simulink model "asbdhc2(1)"  (R2024b)
settings: Solver=ode23  StartTime=0.0  StopTime=100  MaxStep=1/30  RelTol=1e-2  AbsTol=1e-3  EnableMultiTasking=on
PreLoadFcn:
  | load asbdhc2_init;
model workspace (MAT data in the model file):
  op_trim1 = opcond.OperatingReport
  op_trim1.TerminationString_ = '成功满足工作点设定。'
  op_trim1.OptimizationOutput_.iterations = 4
  op_trim1.OptimizationOutput_.funcCount = 131
  op_trim1.OptimizationOutput_.lssteplength = 1
  op_trim1.OptimizationOutput_.stepsize = 7.33681796008e-13
  op_trim1.OptimizationOutput_.algorithm = 'active-set'
  op_trim1.OptimizationOutput_.firstorderopt = 0
  op_trim1.OptimizationOutput_.constrviolation = 7.66053886991e-13
  op_trim1.OptimizationOutput_.message = '找到满足约束的局部最小值。
    | 
    | 优化已完成，因为目标函数沿
    | 可行方向在最优性容差值范围内呈现非递减，
    | 并且在约束容差值范围内满足约束。
    | 
    | <停止条件详细信息>
    | 
    | 优化已完成: 一阶最优性测度 0.000000e+00 小于
    | options.OptimalityTolerance = 1.000000e-06，并且最大约束违反值
    | 7.660539e-13 小于 options.ConstraintTolerance = 1.000000e-06。'
  op_trim1.OptimizationOutput_.bestfeasible.x = [1.78783981281e-13; -2.72791413757e-14; 0.0648890450075; 57.2809333751; -0.648532707323; 3.72213065063; 1.07573812912e-14; 6.1317224328e-16; 3.38561643998e-14; 0; 0; 0; 0; 0; 0; 0; 0; 0; 0; 0; 0; 0; 0; 0; 0; 0; 0; -0.158142456848; -0.114677786174; 0.799732063917; 0.0107264222622]
  op_trim1.OptimizationOutput_.bestfeasible.fval = 0
  op_trim1.OptimizationOutput_.bestfeasible.constrviolation = 7.66053886991e-13
  op_trim1.OptimizationOutput_.bestfeasible.firstorderopt = 0
  op_trim1.OptimizationOutput_.progress = {'<font face="monospaced"; size=3><BR>', '正在优化以求解所有所需的 dx/dt=0、x(k+1)-x(k)=0 和 y=ydes。<BR>', ' <BR>', '(最大误差)模块<BR>', ' ---------------------------------------------------------<BR>', '(1.87100e-01) asbdhc2/De Havilland Beaver Airframe/Aircraft Dynamics/6DOF (Quaternion)/ub,vb,wb<BR>', '(1.25955e-02) asbdhc2/De Havilland Beaver Airframe/Aircraft Dynamics/6DOF (Quaternion)/xe,ye,ze<BR>', '(4.14127e-06) asbdhc2/De Havilland Beaver Airframe/Aircraft Dynamics/6DOF (Quaternion)/xe,ye,ze<BR>', '(7.66054e-13) asbdhc2/De Havilland Beaver Airframe/Aircraft Dynamics/6DOF (Quaternion)/xe,ye,ze<BR>', '(7.66054e-13) asbdhc2/De Havilland Beaver Airframe/Aircraft Dynamics/6DOF (Quaternion)/xe,ye,ze<BR>', ' <BR>', '成功满足工作点设定。<BR>'}
  op_trim1.Model_ = 'asbdhc2'
  op_trim1.States_(1) = opcond.StateReport
  op_trim1.States_(1).dx_ = [0; 0; 0]
  op_trim1.States_(1).Nx_ = 3
  op_trim1.States_(1).Block_ = 'asbdhc2/De Havilland Beaver Airframe/Aircraft Dynamics/6DOF (Quaternion)/Calculate DCM &
    | Euler Angles/phi
    | theta
    | psi'
  op_trim1.States_(1).x_ = [0; 0.0648890450075; 0]
  op_trim1.States_(1).SteadyState_ = [1; 1; 1]
  op_trim1.States_(1).dxMin_ = [-Inf; -Inf; -Inf]
  op_trim1.States_(1).dxMax_ = [Inf; Inf; Inf]
  op_trim1.States_(1).Known_ = [1; 0; 1]
  op_trim1.States_(1).Min_ = [-Inf; -Inf; -Inf]
  op_trim1.States_(1).Max_ = [Inf; Inf; Inf]
  op_trim1.States_(2) = opcond.StateReport
  op_trim1.States_(2).dx_ = [-7.37914856069e-14; 2.85609872713e-14; -2.97018129939e-14]
  op_trim1.States_(2).Nx_ = 3
  op_trim1.States_(2).Block_ = 'asbdhc2/De Havilland Beaver Airframe/Aircraft Dynamics/6DOF (Quaternion)/p,q,r '
  op_trim1.States_(2).x_ = [0; 0; 0]
  op_trim1.States_(2).SteadyState_ = [1; 1; 1]
  op_trim1.States_(2).dxMin_ = [-Inf; -Inf; -Inf]
  op_trim1.States_(2).dxMax_ = [Inf; Inf; Inf]
  op_trim1.States_(2).Known_ = [1; 1; 1]
  op_trim1.States_(2).Min_ = [-Inf; -Inf; -Inf]
  op_trim1.States_(2).Max_ = [Inf; Inf; Inf]
  op_trim1.States_(3) = opcond.StateReport
  op_trim1.States_(3).dx_ = [5.34592169184e-14; -1.7397770363e-13; 2.22581126203e-14]
  op_trim1.States_(3).Nx_ = 3
  op_trim1.States_(3).Block_ = 'asbdhc2/De Havilland Beaver Airframe/Aircraft Dynamics/6DOF (Quaternion)/ub,vb,wb'
  op_trim1.States_(3).x_ = [57.2809333751; -0.648532707323; 3.72213065063]
  op_trim1.States_(3).SteadyState_ = [1; 1; 1]
  op_trim1.States_(3).dxMin_ = [-Inf; -Inf; -Inf]
  op_trim1.States_(3).dxMax_ = [Inf; Inf; Inf]
  op_trim1.States_(3).Known_ = [0; 0; 0]
  op_trim1.States_(3).Min_ = [-Inf; -Inf; -Inf]
  op_trim1.States_(3).Max_ = [Inf; Inf; Inf]
  op_trim1.States_(4) = opcond.StateReport
  op_trim1.States_(4).dx_ = [57.4017385182; -0.648532707323; 7.66053886991e-13]
  op_trim1.States_(4).Nx_ = 3
  op_trim1.States_(4).Block_ = 'asbdhc2/De Havilland Beaver Airframe/Aircraft Dynamics/6DOF (Quaternion)/xe,ye,ze'
  op_trim1.States_(4).x_ = [1.78783981281e-13; -2.72791413757e-14; -50]
  op_trim1.States_(4).SteadyState_ = [0; 0; 1]
  op_trim1.States_(4).dxMin_ = [-Inf; -Inf; -Inf]
  op_trim1.States_(4).dxMax_ = [Inf; Inf; Inf]
  op_trim1.States_(4).Known_ = [0; 0; 1]
  op_trim1.States_(4).Min_ = [-Inf; -Inf; -Inf]
  op_trim1.States_(4).Max_ = [Inf; Inf; Inf]
  op_trim1.States_(5) = opcond.StateReport
  op_trim1.States_(5).Nx_ = 1
  op_trim1.States_(5).Block_ = 'asbdhc2/Environment/Wind Models/Discrete Wind Gust Model/Distance into
    | gust (x)/Distance into
    | Gust (x)
    | (Limited to gust length d)'
  op_trim1.States_(5).SteadyState_ = 0
  op_trim1.States_(5).dxMin_ = -Inf
  op_trim1.States_(5).dxMax_ = Inf
  op_trim1.States_(5).Known_ = 0
  op_trim1.States_(5).Min_ = 0
  op_trim1.States_(5).Max_ = 120
  op_trim1.States_(6) = opcond.StateReport
  op_trim1.States_(6).Nx_ = 1
  op_trim1.States_(6).Block_ = 'asbdhc2/Environment/Wind Models/Discrete Wind Gust Model/Distance into
    | gust (y)/Distance into
    | Gust (x)
    | (Limited to gust length d)
    | '
  op_trim1.States_(6).SteadyState_ = 0
  op_trim1.States_(6).dxMin_ = -Inf
  op_trim1.States_(6).dxMax_ = Inf
  op_trim1.States_(6).Known_ = 0
  op_trim1.States_(6).Min_ = 0
  op_trim1.States_(6).Max_ = 120
  op_trim1.States_(7) = opcond.StateReport
  op_trim1.States_(7).Nx_ = 1
  op_trim1.States_(7).Block_ = 'asbdhc2/Environment/Wind Models/Discrete Wind Gust Model/Distance into
    | gust (z)/Distance into
    | Gust (x)
    | (Limited to gust length d)
    | '
  op_trim1.States_(7).SteadyState_ = 0
  op_trim1.States_(7).dxMin_ = -Inf
  op_trim1.States_(7).dxMax_ = Inf
  op_trim1.States_(7).Known_ = 0
  op_trim1.States_(7).Min_ = 0
  op_trim1.States_(7).Max_ = 80
  op_trim1.States_(8) = opcond.StateReport
  op_trim1.States_(8).dx_ = [0; 0]
  op_trim1.States_(8).Nx_ = 2
  op_trim1.States_(8).Block_ = 'asbdhc2/Environment/Wind Models/Dryden Wind Turbulence Model 
    | (Continuous (+q -r))/Filters on angular rates/Hpgw/pgw_p'
  op_trim1.States_(8).x_ = [0; 0]
  op_trim1.States_(8).SteadyState_ = [0; 0]
  op_trim1.States_(8).dxMin_ = [-Inf; -Inf]
  op_trim1.States_(8).dxMax_ = [Inf; Inf]
  op_trim1.States_(8).Known_ = [0; 0]
  op_trim1.States_(8).Min_ = [-Inf; -Inf]
  op_trim1.States_(8).Max_ = [Inf; Inf]
  op_trim1.States_(9) = opcond.StateReport
  op_trim1.States_(9).dx_ = [0; 0]
  op_trim1.States_(9).Nx_ = 2
  op_trim1.States_(9).Block_ = 'asbdhc2/Environment/Wind Models/Dryden Wind Turbulence Model 
    | (Continuous (+q -r))/Filters on angular rates/Hqgw/qgw_p'
  op_trim1.States_(9).x_ = [0; 0]
  op_trim1.States_(9).SteadyState_ = [0; 0]
  op_trim1.States_(9).dxMin_ = [-Inf; -Inf]
  op_trim1.States_(9).dxMax_ = [Inf; Inf]
  op_trim1.States_(9).Known_ = [0; 0]
  op_trim1.States_(9).Min_ = [-Inf; -Inf]
  op_trim1.States_(9).Max_ = [Inf; Inf]
  op_trim1.States_(10) = opcond.StateReport
  op_trim1.States_(10).dx_ = [0; 0]
  op_trim1.States_(10).Nx_ = 2
  op_trim1.States_(10).Block_ = 'asbdhc2/Environment/Wind Models/Dryden Wind Turbulence Model 
    | (Continuous (+q -r))/Filters on angular rates/Hrgw/rgw_p'
  op_trim1.States_(10).x_ = [0; 0]
  op_trim1.States_(10).SteadyState_ = [0; 0]
  op_trim1.States_(10).dxMin_ = [-Inf; -Inf]
  op_trim1.States_(10).dxMax_ = [Inf; Inf]
  op_trim1.States_(10).Known_ = [0; 0]
  op_trim1.States_(10).Min_ = [-Inf; -Inf]
  op_trim1.States_(10).Max_ = [Inf; Inf]
  op_trim1.States_(11) = opcond.StateReport
  op_trim1.States_(11).dx_ = [0; 0]
  op_trim1.States_(11).Nx_ = 2
  op_trim1.States_(11).Block_ = 'asbdhc2/Environment/Wind Models/Dryden Wind Turbulence Model 
    | (Continuous (+q -r))/Filters on velocities/Hugw(s)/ug_p'
  op_trim1.States_(11).x_ = [0; 0]
  op_trim1.States_(11).SteadyState_ = [0; 0]
  op_trim1.States_(11).dxMin_ = [-Inf; -Inf]
  op_trim1.States_(11).dxMax_ = [Inf; Inf]
  op_trim1.States_(11).Known_ = [0; 0]
  op_trim1.States_(11).Min_ = [-Inf; -Inf]
  op_trim1.States_(11).Max_ = [Inf; Inf]
  op_trim1.States_(12) = opcond.StateReport
  op_trim1.States_(12).dx_ = [0; 0]
  op_trim1.States_(12).Nx_ = 2
  op_trim1.States_(12).Block_ = 'asbdhc2/Environment/Wind Models/Dryden Wind Turbulence Model 
    | (Continuous (+q -r))/Filters on velocities/Hvgw(s)/vg_p1'
  op_trim1.States_(12).x_ = [0; 0]
  op_trim1.States_(12).SteadyState_ = [0; 0]
  op_trim1.States_(12).dxMin_ = [-Inf; -Inf]
  op_trim1.States_(12).dxMax_ = [Inf; Inf]
  op_trim1.States_(12).Known_ = [0; 0]
  op_trim1.States_(12).Min_ = [-Inf; -Inf]
  op_trim1.States_(12).Max_ = [Inf; Inf]
  op_trim1.States_(13) = opcond.StateReport
  op_trim1.States_(13).dx_ = [0; 0]
  op_trim1.States_(13).Nx_ = 2
  op_trim1.States_(13).Block_ = 'asbdhc2/Environment/Wind Models/Dryden Wind Turbulence Model 
    | (Continuous (+q -r))/Filters on velocities/Hvgw(s)/vgw_p2'
  op_trim1.States_(13).x_ = [0; 0]
  op_trim1.States_(13).SteadyState_ = [0; 0]
  op_trim1.States_(13).dxMin_ = [-Inf; -Inf]
  op_trim1.States_(13).dxMax_ = [Inf; Inf]
  op_trim1.States_(13).Known_ = [0; 0]
  op_trim1.States_(13).Min_ = [-Inf; -Inf]
  op_trim1.States_(13).Max_ = [Inf; Inf]
  op_trim1.States_(14) = opcond.StateReport
  op_trim1.States_(14).dx_ = [0; 0]
  op_trim1.States_(14).Nx_ = 2
  op_trim1.States_(14).Block_ = 'asbdhc2/Environment/Wind Models/Dryden Wind Turbulence Model 
    | (Continuous (+q -r))/Filters on velocities/Hwgw(s)/wg_p1'
  op_trim1.States_(14).x_ = [3.38561643998e-14; 0]
  op_trim1.States_(14).SteadyState_ = [0; 0]
  op_trim1.States_(14).dxMin_ = [-Inf; -Inf]
  op_trim1.States_(14).dxMax_ = [Inf; Inf]
  op_trim1.States_(14).Known_ = [0; 0]
  op_trim1.States_(14).Min_ = [-Inf; -Inf]
  op_trim1.States_(14).Max_ = [Inf; Inf]
  op_trim1.States_(15) = opcond.StateReport
  op_trim1.States_(15).dx_ = [0; 0]
  op_trim1.States_(15).Nx_ = 2
  op_trim1.States_(15).Block_ = 'asbdhc2/Environment/Wind Models/Dryden Wind Turbulence Model 
    | (Continuous (+q -r))/Filters on velocities/Hwgw(s)/wg_p2'
  op_trim1.States_(15).x_ = [0; 0]
  op_trim1.States_(15).SteadyState_ = [0; 0]
  op_trim1.States_(15).dxMin_ = [-Inf; -Inf]
  op_trim1.States_(15).dxMax_ = [Inf; Inf]
  op_trim1.States_(15).Known_ = [0; 0]
  op_trim1.States_(15).Min_ = [-Inf; -Inf]
  op_trim1.States_(15).Max_ = [Inf; Inf]
  op_trim1.States_(16) = opcond.StateReport
  op_trim1.States_(16).dx_ = 15.7933119322
  op_trim1.States_(16).Nx_ = 1
  op_trim1.States_(16).Block_ = 'asbdhc2/Subsystem1/Integrator'
  op_trim1.States_(16).x_ = 1.07573812912e-14
  op_trim1.States_(16).SteadyState_ = 0
  op_trim1.States_(16).dxMin_ = -Inf
  op_trim1.States_(16).dxMax_ = Inf
  op_trim1.States_(16).Known_ = 0
  op_trim1.States_(16).Min_ = -Inf
  op_trim1.States_(16).Max_ = Inf
  op_trim1.States_(17) = opcond.StateReport
  op_trim1.States_(17).dx_ = 86.5230923209
  op_trim1.States_(17).Nx_ = 1
  op_trim1.States_(17).Block_ = 'asbdhc2/Subsystem1/Integrator1'
  op_trim1.States_(17).x_ = 6.1317224328e-16
  op_trim1.States_(17).SteadyState_ = 0
  op_trim1.States_(17).dxMin_ = -Inf
  op_trim1.States_(17).dxMax_ = Inf
  op_trim1.States_(17).Known_ = 0
  op_trim1.States_(17).Min_ = -Inf
  op_trim1.States_(17).Max_ = Inf
  op_trim1.Inputs_(1) = opcond.InputReport
  op_trim1.Inputs_(1).Block_ = 'asbdhc2/aileron'
  op_trim1.Inputs_(1).PortWidth_ = 1
  op_trim1.Inputs_(1).PortDimensions_ = [1 1]
  op_trim1.Inputs_(1).u_ = -0.158142456848
  op_trim1.Inputs_(1).Known_ = 0
  op_trim1.Inputs_(1).Min_ = -Inf
  op_trim1.Inputs_(1).Max_ = Inf
  op_trim1.Inputs_(2) = opcond.InputReport
  op_trim1.Inputs_(2).Block_ = 'asbdhc2/elevator'
  op_trim1.Inputs_(2).PortWidth_ = 1
  op_trim1.Inputs_(2).PortDimensions_ = [1 1]
  op_trim1.Inputs_(2).u_ = -0.114677786174
  op_trim1.Inputs_(2).Known_ = 0
  op_trim1.Inputs_(2).Min_ = -Inf
  op_trim1.Inputs_(2).Max_ = Inf
  op_trim1.Inputs_(3) = opcond.InputReport
  op_trim1.Inputs_(3).Block_ = 'asbdhc2/T'
  op_trim1.Inputs_(3).PortWidth_ = 1
  op_trim1.Inputs_(3).PortDimensions_ = [1 1]
  op_trim1.Inputs_(3).u_ = 0.799732063917
  op_trim1.Inputs_(3).Known_ = 0
  op_trim1.Inputs_(3).Min_ = 0
  op_trim1.Inputs_(3).Max_ = 0.8
  op_trim1.Inputs_(4) = opcond.InputReport
  op_trim1.Inputs_(4).Block_ = 'asbdhc2/rudder'
  op_trim1.Inputs_(4).PortWidth_ = 1
  op_trim1.Inputs_(4).PortDimensions_ = [1 1]
  op_trim1.Inputs_(4).u_ = 0.0107264222622
  op_trim1.Inputs_(4).Known_ = 0
  op_trim1.Inputs_(4).Min_ = -Inf
  op_trim1.Inputs_(4).Max_ = Inf
  op_trim2 = opcond.OperatingReport
  op_trim2.TerminationString_ = '成功满足工作点设定。'
  op_trim2.OptimizationOutput_.iterations = 4
  op_trim2.OptimizationOutput_.funcCount = 169
  op_trim2.OptimizationOutput_.lssteplength = 1
  op_trim2.OptimizationOutput_.stepsize = 9.33830695411e-06
  op_trim2.OptimizationOutput_.algorithm = 'active-set'
  op_trim2.OptimizationOutput_.firstorderopt = 1.66504127722e-08
  op_trim2.OptimizationOutput_.constrviolation = 7.19463059795e-10
  op_trim2.OptimizationOutput_.message = '找到满足约束的局部最小值。
    | 
    | 优化已完成，因为目标函数沿
    | 可行方向在最优性容差值范围内呈现非递减，
    | 并且在约束容差值范围内满足约束。
    | 
    | <停止条件详细信息>
    | 
    | 优化已完成: 一阶最优性测度 1.665041e-08 小于
    | options.OptimalityTolerance = 1.000000e-06，并且最大约束违反值
    | 7.194631e-10 小于 options.ConstraintTolerance = 1.000000e-06。'
  op_trim2.OptimizationOutput_.bestfeasible.x = [1.78796394392e-13; -2.74135226799e-14; 0.0648667459691; 57.2818733815; -0.648571858421; 3.72090901022; 1.07573812912e-14; 6.1317224328e-16; 0; 3.38561643998e-14; 0; 0; 0; 0; 0; 0; 0; 0; 0; 0; 0; 0; 0; 0; 0; 0; 0; 0; -0.158142456848; -0.114618135259; 0.423788128522; 0.0167693533563]
  op_trim2.OptimizationOutput_.bestfeasible.fval = 0
  op_trim2.OptimizationOutput_.bestfeasible.constrviolation = 7.19463059795e-10
  op_trim2.OptimizationOutput_.bestfeasible.firstorderopt = 1.66504127722e-08
  op_trim2.OptimizationOutput_.progress = {'<font face="monospaced"; size=3><BR>', '正在优化以求解所有所需的 dx/dt=0、x(k+1)-x(k)=0 和 y=ydes。<BR>', ' <BR>', '(最大误差)模块<BR>', ' ---------------------------------------------------------<BR>', '(3.22464e+00) asbdhc2/De Havilland Beaver Airframe/Aircraft Dynamics/6DOF (Quaternion)/ub,vb,wb<BR>', '(4.57239e-01) asbdhc2/De Havilland Beaver Airframe/Aircraft Dynamics/6DOF (Quaternion)/ub,vb,wb<BR>', '(2.33737e-02) asbdhc2/De Havilland Beaver Airframe/Aircraft Dynamics/6DOF (Quaternion)/ub,vb,wb<BR>', '(7.38836e-05) asbdhc2/De Havilland Beaver Airframe/Aircraft Dynamics/6DOF (Quaternion)/ub,vb,wb<BR>', '(7.19463e-10) asbdhc2/De Havilland Beaver Airframe/Aircraft Dynamics/6DOF (Quaternion)/ub,vb,wb<BR>', '(7.19463e-10) asbdhc2/De Havilland Beaver Airframe/Aircraft Dynamics/6DOF (Quaternion)/ub,vb,wb<BR>', ' <BR>', '成功满足工作点设定。<BR>'}
  op_trim2.Model_ = 'asbdhc2'
  op_trim2.States_(1) = opcond.StateReport
  op_trim2.States_(1).dx_ = [0; 0; 0]
  op_trim2.States_(1).Nx_ = 3
  op_trim2.States_(1).Block_ = 'asbdhc2/De Havilland Beaver Airframe/Aircraft Dynamics/6DOF (Quaternion)/Calculate DCM &
    | Euler Angles/phi
    | theta
    | psi'
  op_trim2.States_(1).x_ = [0; 0.0648667459691; 0]
  op_trim2.States_(1).SteadyState_ = [1; 1; 1]
  op_trim2.States_(1).dxMin_ = [-Inf; -Inf; -Inf]
  op_trim2.States_(1).dxMax_ = [Inf; Inf; Inf]
  op_trim2.States_(1).Known_ = [1; 0; 1]
  op_trim2.States_(1).Min_ = [-Inf; -Inf; -Inf]
  op_trim2.States_(1).Max_ = [Inf; Inf; Inf]
  op_trim2.States_(2) = opcond.StateReport
  op_trim2.States_(2).dx_ = [0; -1.66890739063e-10; 0]
  op_trim2.States_(2).Nx_ = 3
  op_trim2.States_(2).Block_ = 'asbdhc2/De Havilland Beaver Airframe/Aircraft Dynamics/6DOF (Quaternion)/p,q,r '
  op_trim2.States_(2).x_ = [0; 0; 0]
  op_trim2.States_(2).SteadyState_ = [1; 1; 1]
  op_trim2.States_(2).dxMin_ = [-Inf; -Inf; -Inf]
  op_trim2.States_(2).dxMax_ = [Inf; Inf; Inf]
  op_trim2.States_(2).Known_ = [1; 1; 1]
  op_trim2.States_(2).Min_ = [-Inf; -Inf; -Inf]
  op_trim2.States_(2).Max_ = [Inf; Inf; Inf]
  op_trim2.States_(3) = opcond.StateReport
  op_trim2.States_(3).dx_ = [6.98560825185e-10; 0; -7.19463059795e-10]
  op_trim2.States_(3).Nx_ = 3
  op_trim2.States_(3).Block_ = 'asbdhc2/De Havilland Beaver Airframe/Aircraft Dynamics/6DOF (Quaternion)/ub,vb,wb'
  op_trim2.States_(3).x_ = [57.2818733815; -0.648571858421; 3.72090901022]
  op_trim2.States_(3).SteadyState_ = [1; 1; 1]
  op_trim2.States_(3).dxMin_ = [-Inf; -Inf; -Inf]
  op_trim2.States_(3).dxMax_ = [Inf; Inf; Inf]
  op_trim2.States_(3).Known_ = [0; 0; 0]
  op_trim2.States_(3).Min_ = [-Inf; -Inf; -Inf]
  op_trim2.States_(3).Max_ = [Inf; Inf; Inf]
  op_trim2.States_(4) = opcond.StateReport
  op_trim2.States_(4).dx_ = [57.4025973451; -0.648571858421; -1.44328993201e-13]
  op_trim2.States_(4).Nx_ = 3
  op_trim2.States_(4).Block_ = 'asbdhc2/De Havilland Beaver Airframe/Aircraft Dynamics/6DOF (Quaternion)/xe,ye,ze'
  op_trim2.States_(4).x_ = [1.78796394392e-13; -2.74135226799e-14; -50]
  op_trim2.States_(4).SteadyState_ = [0; 0; 1]
  op_trim2.States_(4).dxMin_ = [-Inf; -Inf; -Inf]
  op_trim2.States_(4).dxMax_ = [Inf; Inf; Inf]
  op_trim2.States_(4).Known_ = [0; 0; 1]
  op_trim2.States_(4).Min_ = [-Inf; -Inf; -Inf]
  op_trim2.States_(4).Max_ = [Inf; Inf; Inf]
  op_trim2.States_(5) = opcond.StateReport
  op_trim2.States_(5).Nx_ = 1
  op_trim2.States_(5).Block_ = 'asbdhc2/Environment/Wind Models/Discrete Wind Gust Model/Distance into
    | gust (x)/Distance into
    | Gust (x)
    | (Limited to gust length d)'
  op_trim2.States_(5).SteadyState_ = 0
  op_trim2.States_(5).dxMin_ = -Inf
  op_trim2.States_(5).dxMax_ = Inf
  op_trim2.States_(5).Known_ = 0
  op_trim2.States_(5).Min_ = 0
  op_trim2.States_(5).Max_ = 120
  op_trim2.States_(6) = opcond.StateReport
  op_trim2.States_(6).Nx_ = 1
  op_trim2.States_(6).Block_ = 'asbdhc2/Environment/Wind Models/Discrete Wind Gust Model/Distance into
    | gust (y)/Distance into
    | Gust (x)
    | (Limited to gust length d)
    | '
  op_trim2.States_(6).SteadyState_ = 0
  op_trim2.States_(6).dxMin_ = -Inf
  op_trim2.States_(6).dxMax_ = Inf
  op_trim2.States_(6).Known_ = 0
  op_trim2.States_(6).Min_ = 0
  op_trim2.States_(6).Max_ = 120
  op_trim2.States_(7) = opcond.StateReport
  op_trim2.States_(7).Nx_ = 1
  op_trim2.States_(7).Block_ = 'asbdhc2/Environment/Wind Models/Discrete Wind Gust Model/Distance into
    | gust (z)/Distance into
    | Gust (x)
    | (Limited to gust length d)
    | '
  op_trim2.States_(7).SteadyState_ = 0
  op_trim2.States_(7).dxMin_ = -Inf
  op_trim2.States_(7).dxMax_ = Inf
  op_trim2.States_(7).Known_ = 0
  op_trim2.States_(7).Min_ = 0
  op_trim2.States_(7).Max_ = 80
  op_trim2.States_(8) = opcond.StateReport
  op_trim2.States_(8).dx_ = [0; 0]
  op_trim2.States_(8).Nx_ = 2
  op_trim2.States_(8).Block_ = 'asbdhc2/Environment/Wind Models/Dryden Wind Turbulence Model 
    | (Continuous (+q -r))/Filters on angular rates/Hpgw/pgw_p'
  op_trim2.States_(8).x_ = [0; 0]
  op_trim2.States_(8).SteadyState_ = [0; 0]
  op_trim2.States_(8).dxMin_ = [-Inf; -Inf]
  op_trim2.States_(8).dxMax_ = [Inf; Inf]
  op_trim2.States_(8).Known_ = [0; 0]
  op_trim2.States_(8).Min_ = [-Inf; -Inf]
  op_trim2.States_(8).Max_ = [Inf; Inf]
  op_trim2.States_(9) = opcond.StateReport
  op_trim2.States_(9).dx_ = [0; 0]
  op_trim2.States_(9).Nx_ = 2
  op_trim2.States_(9).Block_ = 'asbdhc2/Environment/Wind Models/Dryden Wind Turbulence Model 
    | (Continuous (+q -r))/Filters on angular rates/Hqgw/qgw_p'
  op_trim2.States_(9).x_ = [0; 0]
  op_trim2.States_(9).SteadyState_ = [0; 0]
  op_trim2.States_(9).dxMin_ = [-Inf; -Inf]
  op_trim2.States_(9).dxMax_ = [Inf; Inf]
  op_trim2.States_(9).Known_ = [0; 0]
  op_trim2.States_(9).Min_ = [-Inf; -Inf]
  op_trim2.States_(9).Max_ = [Inf; Inf]
  op_trim2.States_(10) = opcond.StateReport
  op_trim2.States_(10).dx_ = [0; 0]
  op_trim2.States_(10).Nx_ = 2
  op_trim2.States_(10).Block_ = 'asbdhc2/Environment/Wind Models/Dryden Wind Turbulence Model 
    | (Continuous (+q -r))/Filters on angular rates/Hrgw/rgw_p'
  op_trim2.States_(10).x_ = [0; 0]
  op_trim2.States_(10).SteadyState_ = [0; 0]
  op_trim2.States_(10).dxMin_ = [-Inf; -Inf]
  op_trim2.States_(10).dxMax_ = [Inf; Inf]
  op_trim2.States_(10).Known_ = [0; 0]
  op_trim2.States_(10).Min_ = [-Inf; -Inf]
  op_trim2.States_(10).Max_ = [Inf; Inf]
  op_trim2.States_(11) = opcond.StateReport
  op_trim2.States_(11).dx_ = [0; 0]
  op_trim2.States_(11).Nx_ = 2
  op_trim2.States_(11).Block_ = 'asbdhc2/Environment/Wind Models/Dryden Wind Turbulence Model 
    | (Continuous (+q -r))/Filters on velocities/Hugw(s)/ug_p'
  op_trim2.States_(11).x_ = [0; 0]
  op_trim2.States_(11).SteadyState_ = [0; 0]
  op_trim2.States_(11).dxMin_ = [-Inf; -Inf]
  op_trim2.States_(11).dxMax_ = [Inf; Inf]
  op_trim2.States_(11).Known_ = [0; 0]
  op_trim2.States_(11).Min_ = [-Inf; -Inf]
  op_trim2.States_(11).Max_ = [Inf; Inf]
  op_trim2.States_(12) = opcond.StateReport
  op_trim2.States_(12).dx_ = [0; 0]
  op_trim2.States_(12).Nx_ = 2
  op_trim2.States_(12).Block_ = 'asbdhc2/Environment/Wind Models/Dryden Wind Turbulence Model 
    | (Continuous (+q -r))/Filters on velocities/Hvgw(s)/vg_p1'
  op_trim2.States_(12).x_ = [0; 0]
  op_trim2.States_(12).SteadyState_ = [0; 0]
  op_trim2.States_(12).dxMin_ = [-Inf; -Inf]
  op_trim2.States_(12).dxMax_ = [Inf; Inf]
  op_trim2.States_(12).Known_ = [0; 0]
  op_trim2.States_(12).Min_ = [-Inf; -Inf]
  op_trim2.States_(12).Max_ = [Inf; Inf]
  op_trim2.States_(13) = opcond.StateReport
  op_trim2.States_(13).dx_ = [0; 0]
  op_trim2.States_(13).Nx_ = 2
  op_trim2.States_(13).Block_ = 'asbdhc2/Environment/Wind Models/Dryden Wind Turbulence Model 
    | (Continuous (+q -r))/Filters on velocities/Hvgw(s)/vgw_p2'
  op_trim2.States_(13).x_ = [0; 0]
  op_trim2.States_(13).SteadyState_ = [0; 0]
  op_trim2.States_(13).dxMin_ = [-Inf; -Inf]
  op_trim2.States_(13).dxMax_ = [Inf; Inf]
  op_trim2.States_(13).Known_ = [0; 0]
  op_trim2.States_(13).Min_ = [-Inf; -Inf]
  op_trim2.States_(13).Max_ = [Inf; Inf]
  op_trim2.States_(14) = opcond.StateReport
  op_trim2.States_(14).dx_ = [0; 0]
  op_trim2.States_(14).Nx_ = 2
  op_trim2.States_(14).Block_ = 'asbdhc2/Environment/Wind Models/Dryden Wind Turbulence Model 
    | (Continuous (+q -r))/Filters on velocities/Hwgw(s)/wg_p1'
  op_trim2.States_(14).x_ = [3.38561643998e-14; 0]
  op_trim2.States_(14).SteadyState_ = [0; 0]
  op_trim2.States_(14).dxMin_ = [-Inf; -Inf]
  op_trim2.States_(14).dxMax_ = [Inf; Inf]
  op_trim2.States_(14).Known_ = [0; 0]
  op_trim2.States_(14).Min_ = [-Inf; -Inf]
  op_trim2.States_(14).Max_ = [Inf; Inf]
  op_trim2.States_(15) = opcond.StateReport
  op_trim2.States_(15).dx_ = [0; 0]
  op_trim2.States_(15).Nx_ = 2
  op_trim2.States_(15).Block_ = 'asbdhc2/Environment/Wind Models/Dryden Wind Turbulence Model 
    | (Continuous (+q -r))/Filters on velocities/Hwgw(s)/wg_p2'
  op_trim2.States_(15).x_ = [0; 0]
  op_trim2.States_(15).SteadyState_ = [0; 0]
  op_trim2.States_(15).dxMin_ = [-Inf; -Inf]
  op_trim2.States_(15).dxMax_ = [Inf; Inf]
  op_trim2.States_(15).Known_ = [0; 0]
  op_trim2.States_(15).Min_ = [-Inf; -Inf]
  op_trim2.States_(15).Max_ = [Inf; Inf]
  op_trim2.States_(16) = opcond.StateReport
  op_trim2.States_(16).dx_ = 10.7406261221
  op_trim2.States_(16).Nx_ = 1
  op_trim2.States_(16).Block_ = 'asbdhc2/PID Controller/Integrator/Continuous/Integrator'
  op_trim2.States_(16).SteadyState_ = 0
  op_trim2.States_(16).dxMin_ = -Inf
  op_trim2.States_(16).dxMax_ = Inf
  op_trim2.States_(16).Known_ = 0
  op_trim2.States_(16).Min_ = -Inf
  op_trim2.States_(16).Max_ = Inf
  op_trim2.States_(17) = opcond.StateReport
  op_trim2.States_(17).dx_ = 15.7929765645
  op_trim2.States_(17).Nx_ = 1
  op_trim2.States_(17).Block_ = 'asbdhc2/Subsystem1/Integrator'
  op_trim2.States_(17).x_ = 1.07573812912e-14
  op_trim2.States_(17).SteadyState_ = 0
  op_trim2.States_(17).dxMin_ = -Inf
  op_trim2.States_(17).dxMax_ = Inf
  op_trim2.States_(17).Known_ = 0
  op_trim2.States_(17).Min_ = -Inf
  op_trim2.States_(17).Max_ = Inf
  op_trim2.States_(18) = opcond.StateReport
  op_trim2.States_(18).dx_ = 86.5222922324
  op_trim2.States_(18).Nx_ = 1
  op_trim2.States_(18).Block_ = 'asbdhc2/Subsystem1/Integrator1'
  op_trim2.States_(18).x_ = 6.1317224328e-16
  op_trim2.States_(18).SteadyState_ = 0
  op_trim2.States_(18).dxMin_ = -Inf
  op_trim2.States_(18).dxMax_ = Inf
  op_trim2.States_(18).Known_ = 0
  op_trim2.States_(18).Min_ = -Inf
  op_trim2.States_(18).Max_ = Inf
  op_trim2.Inputs_(1) = opcond.InputReport
  op_trim2.Inputs_(1).Block_ = 'asbdhc2/aileron'
  op_trim2.Inputs_(1).PortWidth_ = 1
  op_trim2.Inputs_(1).PortDimensions_ = [1 1]
  op_trim2.Inputs_(1).u_ = -0.158142456848
  op_trim2.Inputs_(1).Known_ = 0
  op_trim2.Inputs_(1).Min_ = -Inf
  op_trim2.Inputs_(1).Max_ = Inf
  op_trim2.Inputs_(2) = opcond.InputReport
  op_trim2.Inputs_(2).Block_ = 'asbdhc2/elevator'
  op_trim2.Inputs_(2).PortWidth_ = 1
  op_trim2.Inputs_(2).PortDimensions_ = [1 1]
  op_trim2.Inputs_(2).u_ = -0.114618135259
  op_trim2.Inputs_(2).Known_ = 0
  op_trim2.Inputs_(2).Min_ = -Inf
  op_trim2.Inputs_(2).Max_ = Inf
  op_trim2.Inputs_(3) = opcond.InputReport
  op_trim2.Inputs_(3).Block_ = 'asbdhc2/T'
  op_trim2.Inputs_(3).PortWidth_ = 1
  op_trim2.Inputs_(3).PortDimensions_ = [1 1]
  op_trim2.Inputs_(3).u_ = 0.423788128522
  op_trim2.Inputs_(3).Known_ = 0
  op_trim2.Inputs_(3).Min_ = 0
  op_trim2.Inputs_(3).Max_ = 0.6
  op_trim2.Inputs_(4) = opcond.InputReport
  op_trim2.Inputs_(4).Block_ = 'asbdhc2/rudder'
  op_trim2.Inputs_(4).PortWidth_ = 1
  op_trim2.Inputs_(4).PortDimensions_ = [1 1]
  op_trim2.Inputs_(4).u_ = 0.0167693533563
  op_trim2.Inputs_(4).Known_ = 0
  op_trim2.Inputs_(4).Min_ = -Inf
  op_trim2.Inputs_(4).Max_ = Inf
  op_trim3 = opcond.OperatingReport
  op_trim3.TerminationString_ = '成功满足工作点设定。'
  op_trim3.OptimizationOutput_.iterations = 5
  op_trim3.OptimizationOutput_.funcCount = 164
  op_trim3.OptimizationOutput_.lssteplength = 1
  op_trim3.OptimizationOutput_.stepsize = 2.37163847039e-12
  op_trim3.OptimizationOutput_.algorithm = 'active-set'
  op_trim3.OptimizationOutput_.firstorderopt = 0
  op_trim3.OptimizationOutput_.constrviolation = 6.47677497536e-12
  op_trim3.OptimizationOutput_.message = '找到满足约束的局部最小值。
    | 
    | 优化已完成，因为目标函数沿
    | 可行方向在最优性容差值范围内呈现非递减，
    | 并且在约束容差值范围内满足约束。
    | 
    | <停止条件详细信息>
    | 
    | 优化已完成: 一阶最优性测度 0.000000e+00 小于
    | options.OptimalityTolerance = 1.000000e-06，并且最大约束违反值
    | 6.476775e-12 小于 options.ConstraintTolerance = 1.000000e-06。'
  op_trim3.OptimizationOutput_.bestfeasible.x = [2.58857124896e-12; -1.18608434121e-13; 0.110657139935; 46.0358341845; -0.602456435264; 5.1150889011; 5.08548929071e-15; 2.61560883398e-16; 3.38561643998e-14; 0; 0; 0; 0; 0; 0; 0; 0; 0; 0; 0; 0; 0; 0; 0; 0; 0; 0; -0.158099342895; -0.0379410345418; 0.639989610997; 0.0150033657302]
  op_trim3.OptimizationOutput_.bestfeasible.fval = 0
  op_trim3.OptimizationOutput_.bestfeasible.constrviolation = 6.47677497536e-12
  op_trim3.OptimizationOutput_.bestfeasible.firstorderopt = 0
  op_trim3.OptimizationOutput_.progress = {'<font face="monospaced"; size=3><BR>', '正在优化以求解所有所需的 dx/dt=0、x(k+1)-x(k)=0 和 y=ydes。<BR>', ' <BR>', '(最大误差)模块<BR>', ' ---------------------------------------------------------<BR>', '(3.81734e-01) asbdhc2/De Havilland Beaver Airframe/Aircraft Dynamics/6DOF (Quaternion)/ub,vb,wb<BR>', '(4.09324e-01) asbdhc2/De Havilland Beaver Airframe/Aircraft Dynamics/6DOF (Quaternion)/xe,ye,ze<BR>', '(1.74370e-02) asbdhc2/De Havilland Beaver Airframe/Aircraft Dynamics/6DOF (Quaternion)/xe,ye,ze<BR>', '(1.02028e-05) asbdhc2/De Havilland Beaver Airframe/Aircraft Dynamics/6DOF (Quaternion)/xe,ye,ze<BR>', '(6.47677e-12) asbdhc2/De Havilland Beaver Airframe/Aircraft Dynamics/6DOF (Quaternion)/p,q,r <BR>', '(6.47677e-12) asbdhc2/De Havilland Beaver Airframe/Aircraft Dynamics/6DOF (Quaternion)/p,q,r <BR>', ' <BR>', '成功满足工作点设定。<BR>'}
  op_trim3.Model_ = 'asbdhc2'
  op_trim3.States_(1) = opcond.StateReport
  op_trim3.States_(1).dx_ = [0; 0; 0]
  op_trim3.States_(1).Nx_ = 3
  op_trim3.States_(1).Block_ = 'asbdhc2/De Havilland Beaver Airframe/Aircraft Dynamics/6DOF (Quaternion)/Calculate DCM &
    | Euler Angles/phi
    | theta
    | psi'
  op_trim3.States_(1).x_ = [0; 0.110657139935; 0]
  op_trim3.States_(1).SteadyState_ = [1; 1; 1]
  op_trim3.States_(1).dxMin_ = [-Inf; -Inf; -Inf]
  op_trim3.States_(1).dxMax_ = [Inf; Inf; Inf]
  op_trim3.States_(1).Known_ = [1; 0; 1]
  op_trim3.States_(1).Min_ = [-Inf; -Inf; -Inf]
  op_trim3.States_(1).Max_ = [Inf; Inf; Inf]
  op_trim3.States_(2) = opcond.StateReport
  op_trim3.States_(2).dx_ = [1.40985070075e-13; 6.47677497536e-12; -3.92503342732e-14]
  op_trim3.States_(2).Nx_ = 3
  op_trim3.States_(2).Block_ = 'asbdhc2/De Havilland Beaver Airframe/Aircraft Dynamics/6DOF (Quaternion)/p,q,r '
  op_trim3.States_(2).x_ = [0; 0; 0]
  op_trim3.States_(2).SteadyState_ = [1; 1; 1]
  op_trim3.States_(2).dxMin_ = [-Inf; -Inf; -Inf]
  op_trim3.States_(2).dxMax_ = [Inf; Inf; Inf]
  op_trim3.States_(2).Known_ = [1; 1; 1]
  op_trim3.States_(2).Min_ = [-Inf; -Inf; -Inf]
  op_trim3.States_(2).Max_ = [Inf; Inf; Inf]
  op_trim3.States_(3) = opcond.StateReport
  op_trim3.States_(3).dx_ = [2.17811530642e-13; 9.10355048367e-14; 3.64556087417e-12]
  op_trim3.States_(3).Nx_ = 3
  op_trim3.States_(3).Block_ = 'asbdhc2/De Havilland Beaver Airframe/Aircraft Dynamics/6DOF (Quaternion)/ub,vb,wb'
  op_trim3.States_(3).x_ = [46.0358341845; -0.602456435264; 5.1150889011]
  op_trim3.States_(3).SteadyState_ = [1; 1; 1]
  op_trim3.States_(3).dxMin_ = [-Inf; -Inf; -Inf]
  op_trim3.States_(3).dxMax_ = [Inf; Inf; Inf]
  op_trim3.States_(3).Known_ = [0; 0; 0]
  op_trim3.States_(3).Min_ = [-Inf; -Inf; -Inf]
  op_trim3.States_(3).Max_ = [Inf; Inf; Inf]
  op_trim3.States_(4) = opcond.StateReport
  op_trim3.States_(4).dx_ = [46.3191338814; -0.602456435264; -2.34745556327e-12]
  op_trim3.States_(4).Nx_ = 3
  op_trim3.States_(4).Block_ = 'asbdhc2/De Havilland Beaver Airframe/Aircraft Dynamics/6DOF (Quaternion)/xe,ye,ze'
  op_trim3.States_(4).x_ = [2.58857124896e-12; -1.18608434121e-13; -50]
  op_trim3.States_(4).SteadyState_ = [0; 0; 1]
  op_trim3.States_(4).dxMin_ = [-Inf; -Inf; -Inf]
  op_trim3.States_(4).dxMax_ = [Inf; Inf; Inf]
  op_trim3.States_(4).Known_ = [0; 0; 1]
  op_trim3.States_(4).Min_ = [-Inf; -Inf; -Inf]
  op_trim3.States_(4).Max_ = [Inf; Inf; Inf]
  op_trim3.States_(5) = opcond.StateReport
  op_trim3.States_(5).Nx_ = 1
  op_trim3.States_(5).Block_ = 'asbdhc2/Environment/Wind Models/Discrete Wind Gust Model/Distance into
    | gust (x)/Distance into
    | Gust (x)
    | (Limited to gust length d)'
  op_trim3.States_(5).SteadyState_ = 0
  op_trim3.States_(5).dxMin_ = -Inf
  op_trim3.States_(5).dxMax_ = Inf
  op_trim3.States_(5).Known_ = 0
  op_trim3.States_(5).Min_ = 0
  op_trim3.States_(5).Max_ = 120
  op_trim3.States_(6) = opcond.StateReport
  op_trim3.States_(6).Nx_ = 1
  op_trim3.States_(6).Block_ = 'asbdhc2/Environment/Wind Models/Discrete Wind Gust Model/Distance into
    | gust (y)/Distance into
    | Gust (x)
    | (Limited to gust length d)
    | '
  op_trim3.States_(6).SteadyState_ = 0
  op_trim3.States_(6).dxMin_ = -Inf
  op_trim3.States_(6).dxMax_ = Inf
  op_trim3.States_(6).Known_ = 0
  op_trim3.States_(6).Min_ = 0
  op_trim3.States_(6).Max_ = 120
  op_trim3.States_(7) = opcond.StateReport
  op_trim3.States_(7).Nx_ = 1
  op_trim3.States_(7).Block_ = 'asbdhc2/Environment/Wind Models/Discrete Wind Gust Model/Distance into
    | gust (z)/Distance into
    | Gust (x)
    | (Limited to gust length d)
    | '
  op_trim3.States_(7).SteadyState_ = 0
  op_trim3.States_(7).dxMin_ = -Inf
  op_trim3.States_(7).dxMax_ = Inf
  op_trim3.States_(7).Known_ = 0
  op_trim3.States_(7).Min_ = 0
  op_trim3.States_(7).Max_ = 80
  op_trim3.States_(8) = opcond.StateReport
  op_trim3.States_(8).dx_ = [0; 0]
  op_trim3.States_(8).Nx_ = 2
  op_trim3.States_(8).Block_ = 'asbdhc2/Environment/Wind Models/Dryden Wind Turbulence Model 
    | (Continuous (+q -r))/Filters on angular rates/Hpgw/pgw_p'
  op_trim3.States_(8).x_ = [0; 0]
  op_trim3.States_(8).SteadyState_ = [0; 0]
  op_trim3.States_(8).dxMin_ = [-Inf; -Inf]
  op_trim3.States_(8).dxMax_ = [Inf; Inf]
  op_trim3.States_(8).Known_ = [0; 0]
  op_trim3.States_(8).Min_ = [-Inf; -Inf]
  op_trim3.States_(8).Max_ = [Inf; Inf]
  op_trim3.States_(9) = opcond.StateReport
  op_trim3.States_(9).dx_ = [0; 0]
  op_trim3.States_(9).Nx_ = 2
  op_trim3.States_(9).Block_ = 'asbdhc2/Environment/Wind Models/Dryden Wind Turbulence Model 
    | (Continuous (+q -r))/Filters on angular rates/Hqgw/qgw_p'
  op_trim3.States_(9).x_ = [0; 0]
  op_trim3.States_(9).SteadyState_ = [0; 0]
  op_trim3.States_(9).dxMin_ = [-Inf; -Inf]
  op_trim3.States_(9).dxMax_ = [Inf; Inf]
  op_trim3.States_(9).Known_ = [0; 0]
  op_trim3.States_(9).Min_ = [-Inf; -Inf]
  op_trim3.States_(9).Max_ = [Inf; Inf]
  op_trim3.States_(10) = opcond.StateReport
  op_trim3.States_(10).dx_ = [0; 0]
  op_trim3.States_(10).Nx_ = 2
  op_trim3.States_(10).Block_ = 'asbdhc2/Environment/Wind Models/Dryden Wind Turbulence Model 
    | (Continuous (+q -r))/Filters on angular rates/Hrgw/rgw_p'
  op_trim3.States_(10).x_ = [0; 0]
  op_trim3.States_(10).SteadyState_ = [0; 0]
  op_trim3.States_(10).dxMin_ = [-Inf; -Inf]
  op_trim3.States_(10).dxMax_ = [Inf; Inf]
  op_trim3.States_(10).Known_ = [0; 0]
  op_trim3.States_(10).Min_ = [-Inf; -Inf]
  op_trim3.States_(10).Max_ = [Inf; Inf]
  op_trim3.States_(11) = opcond.StateReport
  op_trim3.States_(11).dx_ = [0; 0]
  op_trim3.States_(11).Nx_ = 2
  op_trim3.States_(11).Block_ = 'asbdhc2/Environment/Wind Models/Dryden Wind Turbulence Model 
    | (Continuous (+q -r))/Filters on velocities/Hugw(s)/ug_p'
  op_trim3.States_(11).x_ = [0; 0]
  op_trim3.States_(11).SteadyState_ = [0; 0]
  op_trim3.States_(11).dxMin_ = [-Inf; -Inf]
  op_trim3.States_(11).dxMax_ = [Inf; Inf]
  op_trim3.States_(11).Known_ = [0; 0]
  op_trim3.States_(11).Min_ = [-Inf; -Inf]
  op_trim3.States_(11).Max_ = [Inf; Inf]
  op_trim3.States_(12) = opcond.StateReport
  op_trim3.States_(12).dx_ = [0; 0]
  op_trim3.States_(12).Nx_ = 2
  op_trim3.States_(12).Block_ = 'asbdhc2/Environment/Wind Models/Dryden Wind Turbulence Model 
    | (Continuous (+q -r))/Filters on velocities/Hvgw(s)/vg_p1'
  op_trim3.States_(12).x_ = [0; 0]
  op_trim3.States_(12).SteadyState_ = [0; 0]
  op_trim3.States_(12).dxMin_ = [-Inf; -Inf]
  op_trim3.States_(12).dxMax_ = [Inf; Inf]
  op_trim3.States_(12).Known_ = [0; 0]
  op_trim3.States_(12).Min_ = [-Inf; -Inf]
  op_trim3.States_(12).Max_ = [Inf; Inf]
  op_trim3.States_(13) = opcond.StateReport
  op_trim3.States_(13).dx_ = [0; 0]
  op_trim3.States_(13).Nx_ = 2
  op_trim3.States_(13).Block_ = 'asbdhc2/Environment/Wind Models/Dryden Wind Turbulence Model 
    | (Continuous (+q -r))/Filters on velocities/Hvgw(s)/vgw_p2'
  op_trim3.States_(13).x_ = [0; 0]
  op_trim3.States_(13).SteadyState_ = [0; 0]
  op_trim3.States_(13).dxMin_ = [-Inf; -Inf]
  op_trim3.States_(13).dxMax_ = [Inf; Inf]
  op_trim3.States_(13).Known_ = [0; 0]
  op_trim3.States_(13).Min_ = [-Inf; -Inf]
  op_trim3.States_(13).Max_ = [Inf; Inf]
  op_trim3.States_(14) = opcond.StateReport
  op_trim3.States_(14).dx_ = [0; 0]
  op_trim3.States_(14).Nx_ = 2
  op_trim3.States_(14).Block_ = 'asbdhc2/Environment/Wind Models/Dryden Wind Turbulence Model 
    | (Continuous (+q -r))/Filters on velocities/Hwgw(s)/wg_p1'
  op_trim3.States_(14).x_ = [3.38561643998e-14; 0]
  op_trim3.States_(14).SteadyState_ = [0; 0]
  op_trim3.States_(14).dxMin_ = [-Inf; -Inf]
  op_trim3.States_(14).dxMax_ = [Inf; Inf]
  op_trim3.States_(14).Known_ = [0; 0]
  op_trim3.States_(14).Min_ = [-Inf; -Inf]
  op_trim3.States_(14).Max_ = [Inf; Inf]
  op_trim3.States_(15) = opcond.StateReport
  op_trim3.States_(15).dx_ = [0; 0]
  op_trim3.States_(15).Nx_ = 2
  op_trim3.States_(15).Block_ = 'asbdhc2/Environment/Wind Models/Dryden Wind Turbulence Model 
    | (Continuous (+q -r))/Filters on velocities/Hwgw(s)/wg_p2'
  op_trim3.States_(15).x_ = [0; 0]
  op_trim3.States_(15).SteadyState_ = [0; 0]
  op_trim3.States_(15).dxMin_ = [-Inf; -Inf]
  op_trim3.States_(15).dxMax_ = [Inf; Inf]
  op_trim3.States_(15).Known_ = [0; 0]
  op_trim3.States_(15).Min_ = [-Inf; -Inf]
  op_trim3.States_(15).Max_ = [Inf; Inf]
  op_trim3.States_(16) = opcond.StateReport
  op_trim3.States_(16).dx_ = 20.8833468134
  op_trim3.States_(16).Nx_ = 1
  op_trim3.States_(16).Block_ = 'asbdhc2/Subsystem1/Integrator'
  op_trim3.States_(16).x_ = 5.08548929071e-15
  op_trim3.States_(16).SteadyState_ = 0
  op_trim3.States_(16).dxMin_ = -Inf
  op_trim3.States_(16).dxMax_ = Inf
  op_trim3.States_(16).Known_ = 0
  op_trim3.States_(16).Min_ = -Inf
  op_trim3.States_(16).Max_ = Inf
  op_trim3.States_(17) = opcond.StateReport
  op_trim3.States_(17).dx_ = 100.664745989
  op_trim3.States_(17).Nx_ = 1
  op_trim3.States_(17).Block_ = 'asbdhc2/Subsystem1/Integrator1'
  op_trim3.States_(17).x_ = 2.61560883398e-16
  op_trim3.States_(17).SteadyState_ = 0
  op_trim3.States_(17).dxMin_ = -Inf
  op_trim3.States_(17).dxMax_ = Inf
  op_trim3.States_(17).Known_ = 0
  op_trim3.States_(17).Min_ = -Inf
  op_trim3.States_(17).Max_ = Inf
  op_trim3.Inputs_(1) = opcond.InputReport
  op_trim3.Inputs_(1).Block_ = 'asbdhc2/aileron'
  op_trim3.Inputs_(1).PortWidth_ = 1
  op_trim3.Inputs_(1).PortDimensions_ = [1 1]
  op_trim3.Inputs_(1).u_ = -0.158099342895
  op_trim3.Inputs_(1).Known_ = 0
  op_trim3.Inputs_(1).Min_ = -Inf
  op_trim3.Inputs_(1).Max_ = Inf
  op_trim3.Inputs_(2) = opcond.InputReport
  op_trim3.Inputs_(2).Block_ = 'asbdhc2/elevator'
  op_trim3.Inputs_(2).PortWidth_ = 1
  op_trim3.Inputs_(2).PortDimensions_ = [1 1]
  op_trim3.Inputs_(2).u_ = -0.0379410345418
  op_trim3.Inputs_(2).Known_ = 0
  op_trim3.Inputs_(2).Min_ = -Inf
  op_trim3.Inputs_(2).Max_ = Inf
  op_trim3.Inputs_(3) = opcond.InputReport
  op_trim3.Inputs_(3).Block_ = 'asbdhc2/T'
  op_trim3.Inputs_(3).PortWidth_ = 1
  op_trim3.Inputs_(3).PortDimensions_ = [1 1]
  op_trim3.Inputs_(3).u_ = 0.639989610997
  op_trim3.Inputs_(3).Known_ = 0
  op_trim3.Inputs_(3).Min_ = 0.5
  op_trim3.Inputs_(3).Max_ = 0.64
  op_trim3.Inputs_(4) = opcond.InputReport
  op_trim3.Inputs_(4).Block_ = 'asbdhc2/rudder'
  op_trim3.Inputs_(4).PortWidth_ = 1
  op_trim3.Inputs_(4).PortDimensions_ = [1 1]
  op_trim3.Inputs_(4).u_ = 0.0150033657302
  op_trim3.Inputs_(4).Known_ = 0
  op_trim3.Inputs_(4).Min_ = -Inf
  op_trim3.Inputs_(4).Max_ = Inf
values from neighbouring files (symbols this model uses):
  beaver_b = 14.63    [aero.mat]
  beaver_c = 1.5875    [aero.mat]
  beaver_init_p = 0    [aero.mat]
  beaver_init_q = 0    [aero.mat]
  beaver_init_r = 0    [aero.mat]
  beaver_init_roll = 0    [aero.mat]
  beaver_mass = 2288.231    [aero.mat]
  Cl_alpha2_dpt = -0.01406    [aero.mat]
  Cl_beta = -0.0618    [aero.mat]
  Cl_da = -0.09917    [aero.mat]
  Cl_da_alpha = -0.08269    [aero.mat]
  Cl_dr = 0.006934    [aero.mat]
  Cl_p = -0.5045    [aero.mat]
  Cl_r = 0.1695    [aero.mat]
  Cm0 = 0.09448    [aero.mat]
  Cm_alpha = -0.6028    [aero.mat]
  Cm_alpha2 = -2.14    [aero.mat]
  Cm_beta2 = 0.6921    [aero.mat]
  Cm_de = -1.921    [aero.mat]
  Cm_df = 0.4072    [aero.mat]
  Cm_dpt = -0.07895    [aero.mat]
  Cm_q = -15.56    [aero.mat]
  Cm_r = -0.3118    [aero.mat]
  Cn_beta = 0.006719    [aero.mat]
  Cn_beta3 = 0.1373    [aero.mat]
  Cn_da = -0.003872    [aero.mat]
  Cn_dpt3 = -0.003026    [aero.mat]
  Cn_dr = -0.08265    [aero.mat]
  Cn_p = -0.1585    [aero.mat]
  Cn_q = 0.1595    [aero.mat]
  Cn_r = -0.1112    [aero.mat]
  Cx0 = -0.03554    [aero.mat]
  Cx_alpha = 0.00292    [aero.mat]
  Cx_alpha2 = 5.459    [aero.mat]
  Cx_alpha3 = -5.162    [aero.mat]
  Cx_df = -0.09447    [aero.mat]
  Cx_df_alpha = 1.106    [aero.mat]
  Cx_dpt = 0.1161    [aero.mat]
  Cx_dpt2_alpha = 0.1453    [aero.mat]
  Cx_dr = 0.03412    [aero.mat]
  Cx_q = -0.6748    [aero.mat]
  Cy0 = -0.002226    [aero.mat]
  Cy_beta = -0.7678    [aero.mat]
  Cy_da = -0.02956    [aero.mat]
  Cy_dr = 0.1158    [aero.mat]
  Cy_dr_alpha = 0.5238    [aero.mat]
  Cy_p = -0.124    [aero.mat]
  Cy_r = 0.3666    [aero.mat]
  Cz0 = -0.05504    [aero.mat]
  Cz_alpha = -5.578    [aero.mat]
  Cz_alpha3 = 3.442    [aero.mat]
  Cz_de = -0.398    [aero.mat]
  Cz_de_beta = -15.93    [aero.mat]
  Cz_df = -1.377    [aero.mat]
  Cz_df_alpha = -1.261    [aero.mat]
  Cz_dpt = -0.1563    [aero.mat]
  Cz_q = -2.988    [aero.mat]
  uaero0 = [-0.0317656979071 -0.0320210159663 -0.0365180369264 0]    [aero.mat]
undefined symbols (not defined in the file or in its folder): Earth, F, Light, MIL, Receive, report2, Send, WGS84
libraries: aerolibconvert2 x3, aerolibwind2 x3, slpidlib x3, aerolibasang x2, aerolibfltsims x2, aerolibanimutils x2, shared6dof x1, aerolibadyn x1, aerolibatmos2 x1, simulink x1, aerolibtransform2 x1
(part 1 of 2)
Description:
  | Fly the De Havilland Beaver
  | 
  | This example uses a pilot's joystick to allow you to fly the De Havilland
  | Beaver modeled with Simulink(R) and Aerospace Blockset(TM) software.
  | This model has been color coded to aid in locating Aerospace Blockset blocks.
  | The red blocks are Aerospace Blockset blocks, the orange blocks are subsystems
  | containing additional Aerospace Blockset blocks and the white blocks are Simulink
  | blocks.
  | 
  | The De Havilland Beaver model includes the airframe dynamics, including
  | aerodynamics. Effects of the environment are also modeled, such as wind profiles
  | for the landing phase. Visualization for this model is done via an interface to
  | FlightGear, a open source flight simulator package.
  | 
  | The De Havilland Beaver was first flown in 1947. Today it is still prized by pilots
  | for its reliability and versatility. The De Havilland Beaver can be operated on wheels,
  | skis or float landing gear.
  | 
  | Speed Max       110 kts
  | Altitude Max 10,000 ft
  | Range Max       400 nm
  | Load                     6 passengers
  | Crew                     1 member
  | 
  | For more information on the FlightGear interface, see the documentation.
settings Model: Creator=The MathWorks, Inc.  LastModifiedBy=22306
settings SolverCC: AutoScaleAbsTol=off  AlgebraicLoopSolver=TrustRegion
settings DataIOCC: ExternalInput=getinputstruct(op_trim2)  InitialState=getstatestruct(op_trim2)  LoadExternalInput=on  LoadInitialState=on  SaveFormat=Array  ReturnWorkspaceOutputs=off  SignalLoggingName=sigsOut
settings OptimizationCC: DefaultParameterBehavior=Inlined  InlineInvariantSignals=on  ExpressionDepthLimit=2147483647  InitFltsAndDblsToZero=on  EfficientFloat2IntCast=on  EfficientMapNaN2IntZero=off  LifeSpan=inf
settings DebuggingCC: MultiTaskCondExecSysMsg=none  SigSpecEnsureSampleTimeMsg=none  IntegerOverflowMsg=none  FcnCallInpInsideContextMsg=warning  UnconnectedInputMsg=warning  UnconnectedOutputMsg=warning  UnconnectedLineMsg=warning  UniqueDataStoreMsg=error  AllowSymbolicDim=off  StateNameClashWarn=warning  StrictBusMsg=ErrorOnBusTreatedAsVector  SFUnexpectedBacktrackingDiag=warning  SFNoUnconditionalDefaultTransitionDiag=warning  SFExecutionAtInitializationDiag=none  IntegerSaturationMsg=none  ArithmeticOperatorsInVariantConditions=warning
settings HardwareCC: ProdBitPerPointer=32  ProdBitPerSizeT=32  ProdBitPerPtrDiffT=32  ProdLargestAtomicFloat=None  ProdIntDivRoundTo=Undefined  ProdEndianess=Unspecified  ProdWordSize=32  ProdHWDeviceType=32-bit Generic  TargetBitPerPointer=64  TargetBitPerSizeT=64  TargetBitPerPtrDiffT=64  TargetLongLongMode=on  TargetIntDivRoundTo=Zero  TargetEndianess=LittleEndian  TargetWordSize=64  TargetHWDeviceType=MATLAB Host  ProdEqTarget=off
settings ModelReferenceCC: EnableRefExpFcnMdlSchedulingChecks=on  PropagateSignalLabelsOutOfModel=off
settings SFSimCC: SimUseLocalCustomCode=off  CustomCodeUndefinedFunction=UseInterfaceOnly
settings RTWCC: RTWUseLocalCustomCode=off  GPUComputeCapability=3.5
settings CodeAppCC: StateflowObjectComments=on
settings GRTTargetCC: TargetFcnLib=ansi_tfl_tmw.mat  TargetLangStandard=C89/C90 (ANSI)  CombineOutputUpdateFcns=off  GRTInterface=on
settings ConfigComp: CovMetricSettings=dw  CovSaveCumulativeToWorkspaceVar=on  CovSaveSingleToWorkspaceVar=on  CovExternalEMLEnable=off  CovSFcnEnable=off

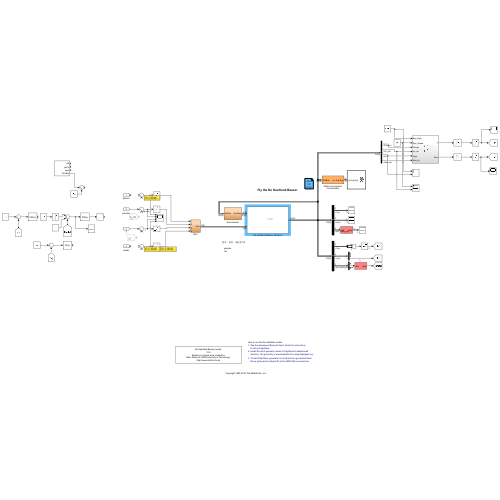
[thumbnail: Simulink's stored preview of the top-level diagram]
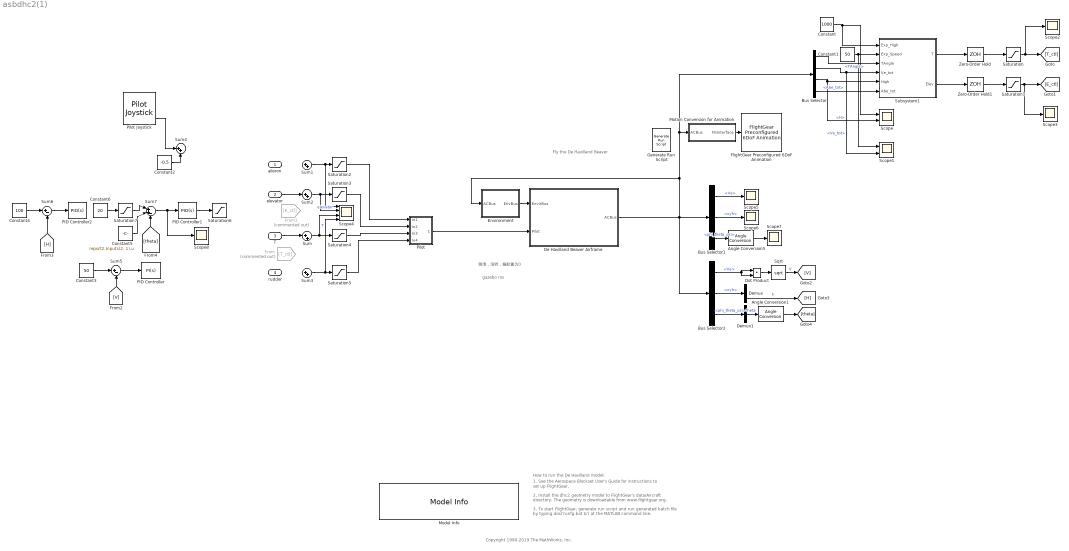
== system asbdhc2(1) ==
  note: gazebo
      | ros
  note: 侧滑，滚转，偏航置为0
  note: 1. See the Aerospace Blockset User's Guide for instructions
      |     to set up FlightGear.
  note: Copyright 1990-2019 The MathWorks, Inc.
  note: Fly the De Havilland Beaver
  note: 2. Install the dhc2 geometry model to FlightGear's data/Aircraft
      |     directory. The geometry is downloadable from www.flightgear.org.
  note: 3. To start FlightGear, generate run script and run generated batch
      |     file by typing dos('runfg.bat &') at the MATLAB command line.
  note: How to run the De Havilland model:
  aileron : Inport
  elevator : Inport  Port=2
  T : Inport  Port=3
  rudder : Inport  Port=4
  Angle Conversion1 : aerolibconvert2/Angle Conversion  IU=rad  OU=deg
  Angle Conversion5 : aerolibconvert2/Angle Conversion  IU=rad  OU=deg
  Bus Selector : BusSelector  OutputSignals=TAngle,Ve_tot,H,Abe_tot
  Bus Selector1 : BusSelector  OutputSignals=Ve,xyh,phi_theta_psi
  Bus Selector2 : BusSelector  OutputSignals=Ve,xyh,phi_theta_psi
  Constant : Constant  Value=1000
  Constant1 : Constant  Value=50
  Constant2 : Constant  Value=-0.5
  Constant3 : Constant  Value=50
  Constant4 : Constant  Value=100
  Constant5 : Constant  Value=report2.Inputs(2, 1).u
  Constant6 : Constant  Value=20
  De Havilland Beaver Airframe : Subsystem
      mask Display: image('asbbeaver.jpg')
  Demux : Demux  Outputs=3
  Demux1 : Demux  Outputs=3
  Dot Product : DotProduct  OutDataTypeStr=Inherit: Inherit via internal rule
  Environment : Subsystem
  FlightGear Preconfigured 6DoF Animation : aerolibfltsims/FlightGear Preconfigured 6DoF Animation  xFlightGearVersion=v2019.1  DestinationIpAddress=127.0.0.1  DestinationPort=5502  SampleTime=1/30  packetVersion=24
  From : From  Commented=on  GotoTag=T_ctl
  From1 : From  Commented=on  GotoTag=E_ctl
  Generate Run Script : aerolibfltsims/Generate Run Script  Architecture=Win64  dataFlow=Send-Receive  GeometryModelName=c172p  AirportId=KSFO  RunwayId=10L  InitialAltitude=7224  InitialHeading=113  OffsetDistance=4.72  OffsetAzimuth=0  InstallScenery=off  DisableShaders=off  OriginAddress=127.0.0.1  DestinationPort=5502  OriginPort=5505  LocalAddress=127.0.0.1  OutputFileName=runfg.bat  FlightGearBaseDirectory=C:\Program Files\FlightGear 2020.3
  Model Info : simulink/Model-Wide Utilities/Model Info  Frame=on  DisplayStringWithTags=|  HorizontalTextAlignment=Center  LeftAlignmentValue=0.5
      | De Havilland Beaver model 
      | %<ModelVersion>
      | Based on original work created by
      | Marc Rauw for Delft University of Technology 
      | http://www.dutchroll.com
  Motion Conversion for Animation : Subsystem
      mask Display:
      | port_label('input',1,'ACBus')
      | port_label('output',1,'\lambda,L,h,\phi,\theta,\psi','texmode','on')
  PID Controller : slpidlib/PID Controller  Controller=PI  Form=Parallel  TimeDomain=Continuous-time  UseExternalTs=off  SampleTime=-1  IntegratorMethod=Forward Euler  FilterMethod=Forward Euler  ControllerParametersSource=internal  P=0.1  I=0.1  UseKiTs=off  D=413.597915956416  UseExternalDerivativeSource=off  N=0.00856107780449433  UseFilter=on  TunerSelectOption=Transfer Function Based (PID Tuner App)  InitialConditionSource=internal  InitialConditionForIntegrator=0  InitialConditionForFilter=0  DifferentiatorICPrevScaledInput=0  ExternalReset=none  TrackingMode=off  Kt=1  LimitOutput=off  SatLimitsSource=internal  UpperSaturationLimit=inf  LowerSaturationLimit=-inf  LinearizeAsGain=on  AntiWindupMode=none  Kb=1  LimitIntegrator=off  UpperIntegratorSaturationLimit=inf  LowerIntegratorSaturationLimit=-inf  POutMin=[]  POutMax=[]  IOutMin=[]  IOutMax=[]  DOutMin=[]  DOutMax=[]  NOutMin=[]  NOutMax=[]  SumOutMin=[]  SumOutMax=[]  SaturationOutMin=[]  SaturationOutMax=[]  PParamMin=[]  PParamMax=[]  IParamMin=[]  IParamMax=[]  DParamMin=[]  DParamMax=[]  NParamMin=[]  NParamMax=[]  KbParamMin=[]  KbParamMax=[]  KtParamMin=[]  KtParamMax=[]  KbOutMin=[]  KbOutMax=[]  KtOutMin=[]  KtOutMax=[]  IntegratorOutMin=[]  IntegratorOutMax=[]  FilterOutMin=[]  FilterOutMax=[]  SumI1OutMin=[]  SumI1OutMax=[]  SumI2OutMin=[]  SumI2OutMax=[]  SumI3OutMin=[]  SumI3OutMax=[]  SumI4OutMin=[]  SumI4OutMax=[]  SumDOutMin=[]  SumDOutMax=[]  DifferentiatorOutMin=[]  DifferentiatorOutMax=[]  FilterDiffOutCoefMin=[]  FilterDiffOutCoefMax=[]  ReciprocalOutMin=[]  ReciprocalOutMax=[]  SumDenOutMin=[]  SumDenOutMax=[]  SumNumOutMin=[]  SumNumOutMax=[]  DivideOutMin=[]  DivideOutMax=[]  UdiffTsProdOutMin=[]  UdiffTsProdOutMax=[]  NTsProdOutMin=[]  NTsProdOutMax=[]  UintegralTsProdOutMin=[]  UintegralTsProdOutMax=[]  UngainTsProdOutMin=[]  UngainTsProdOutMax=[]  ClampingZeroOutDataTypeStr=Inherit: Inherit via back propagation  ClampingZeroOutMin=[]  ClampingZeroOutMax=[]  FilterDenConstantOutDataTypeStr=Inherit: Inherit via back propagation  FilterDenConstantOutMin=[]  FilterDenConstantOutMax=[]  PCopyOutDataTypeStr=Inherit: Inherit via back propagation  PCopyOutMin=[]  PCopyOutMax=[]  NCopyOutDataTypeStr=Inherit: Inherit via back propagation  NCopyOutMin=[]  NCopyOutMax=[]  IntegratorContinuousStateAttributes=''  IntegratorStateMustResolveToSignalObject=off  IntegratorRTWStateStorageClass=Auto  FilterContinuousStateAttributes=''  FilterStateMustResolveToSignalObject=off  FilterRTWStateStorageClass=Auto  ParallelPVariant=InternalParameters  IdealPVariant=Disabled  IVariant=InternalParameters  DVariant=Disabled  IntegratorVariant=Continuous  SatVariant=Disabled  AWVariant=Passthrough  PCopyVariant=Disabled  TRVariant=Disabled  FdbkBlocksVariant=Forward  IdealPFdbkVariant=Disabled  SatFdbkVariant=Disabled  DerivativeFilterVariant=Disabled  NVariant=Disabled  NCopyVariant=Disabled_SignalSpec  FilterICVariant=Disabled  IntegratorICVariant=InternalICs  ExternalResetVariant=Disabled  TRSumVariant=Passthrough  SumFdbkVariant=Disabled  SumVariant=Sum_PI  TsampFilterVariant=InternalTs  TsampNgainVariant=Passthrough  TsampIntegralVariant=Disabled_SignalSpec  ExternalSaturationOutDataTypeStr=Inherit: Same as second input  DerivativeSourceVariant=Disabled  PreIntVariant=InternalPreInt
  PID Controller1 : slpidlib/PID Controller  Controller=PID  Form=Parallel  TimeDomain=Continuous-time  UseExternalTs=off  SampleTime=-1  IntegratorMethod=Forward Euler  FilterMethod=Forward Euler  ControllerParametersSource=internal  P=0.5  I=0  UseKiTs=off  D=5  UseExternalDerivativeSource=off  N=100  UseFilter=on  TunerSelectOption=Transfer Function Based (PID Tuner App)  InitialConditionSource=internal  InitialConditionForIntegrator=0  InitialConditionForFilter=0  DifferentiatorICPrevScaledInput=0  ExternalReset=none  TrackingMode=off  Kt=1  LimitOutput=off  SatLimitsSource=internal  UpperSaturationLimit=inf  LowerSaturationLimit=-inf  LinearizeAsGain=on  AntiWindupMode=none  Kb=1  LimitIntegrator=off  UpperIntegratorSaturationLimit=inf  LowerIntegratorSaturationLimit=-inf  POutMin=[]  POutMax=[]  IOutMin=[]  IOutMax=[]  DOutMin=[]  DOutMax=[]  NOutMin=[]  NOutMax=[]  SumOutMin=[]  SumOutMax=[]  SaturationOutMin=[]  SaturationOutMax=[]  PParamMin=[]  PParamMax=[]  IParamMin=[]  IParamMax=[]  DParamMin=[]  DParamMax=[]  NParamMin=[]  NParamMax=[]  KbParamMin=[]  KbParamMax=[]  KtParamMin=[]  KtParamMax=[]  KbOutMin=[]  KbOutMax=[]  KtOutMin=[]  KtOutMax=[]  IntegratorOutMin=[]  IntegratorOutMax=[]  FilterOutMin=[]  FilterOutMax=[]  SumI1OutMin=[]  SumI1OutMax=[]  SumI2OutMin=[]  SumI2OutMax=[]  SumI3OutMin=[]  SumI3OutMax=[]  SumI4OutMin=[]  SumI4OutMax=[]  SumDOutMin=[]  SumDOutMax=[]  DifferentiatorOutMin=[]  DifferentiatorOutMax=[]  FilterDiffOutCoefMin=[]  FilterDiffOutCoefMax=[]  ReciprocalOutMin=[]  ReciprocalOutMax=[]  SumDenOutMin=[]  SumDenOutMax=[]  SumNumOutMin=[]  SumNumOutMax=[]  DivideOutMin=[]  DivideOutMax=[]  UdiffTsProdOutMin=[]  UdiffTsProdOutMax=[]  NTsProdOutMin=[]  NTsProdOutMax=[]  UintegralTsProdOutMin=[]  UintegralTsProdOutMax=[]  UngainTsProdOutMin=[]  UngainTsProdOutMax=[]  ClampingZeroOutDataTypeStr=Inherit: Inherit via back propagation  ClampingZeroOutMin=[]  ClampingZeroOutMax=[]  FilterDenConstantOutDataTypeStr=Inherit: Inherit via back propagation  FilterDenConstantOutMin=[]  FilterDenConstantOutMax=[]  PCopyOutDataTypeStr=Inherit: Inherit via back propagation  PCopyOutMin=[]  PCopyOutMax=[]  NCopyOutDataTypeStr=Inherit: Inherit via back propagation  NCopyOutMin=[]  NCopyOutMax=[]  IntegratorContinuousStateAttributes=''  IntegratorStateMustResolveToSignalObject=off  IntegratorRTWStateStorageClass=Auto  FilterContinuousStateAttributes=''  FilterStateMustResolveToSignalObject=off  FilterRTWStateStorageClass=Auto  ParallelPVariant=InternalParameters  IdealPVariant=Disabled  IVariant=InternalParameters  DVariant=InternalParameters  IntegratorVariant=Continuous  SatVariant=Disabled  AWVariant=Passthrough  PCopyVariant=Disabled  TRVariant=Disabled  FdbkBlocksVariant=Forward  IdealPFdbkVariant=Disabled  SatFdbkVariant=Disabled  DerivativeFilterVariant=ContFilter  NVariant=InternalParameters  NCopyVariant=Disabled  FilterICVariant=InternalICsFilter  IntegratorICVariant=InternalICs  ExternalResetVariant=Disabled  TRSumVariant=Passthrough  SumFdbkVariant=Disabled  SumVariant=Sum_PID  TsampFilterVariant=InternalTs  TsampNgainVariant=Passthrough  TsampIntegralVariant=Disabled_SignalSpec  ExternalSaturationOutDataTypeStr=Inherit: Same as second input  DerivativeSourceVariant=ErrorSignal  PreIntVariant=InternalPreInt
  PID Controller2 : slpidlib/PID Controller  Controller=PID  Form=Parallel  TimeDomain=Continuous-time  UseExternalTs=off  SampleTime=-1  IntegratorMethod=Forward Euler  FilterMethod=Forward Euler  ControllerParametersSource=internal  P=1  I=1  UseKiTs=off  D=0  UseExternalDerivativeSource=off  N=100  UseFilter=on  TunerSelectOption=Transfer Function Based (PID Tuner App)  InitialConditionSource=internal  InitialConditionForIntegrator=0  InitialConditionForFilter=0  DifferentiatorICPrevScaledInput=0  ExternalReset=none  TrackingMode=off  Kt=1  LimitOutput=off  SatLimitsSource=internal  UpperSaturationLimit=inf  LowerSaturationLimit=-inf  LinearizeAsGain=on  AntiWindupMode=none  Kb=1  LimitIntegrator=off  UpperIntegratorSaturationLimit=inf  LowerIntegratorSaturationLimit=-inf  POutMin=[]  POutMax=[]  IOutMin=[]  IOutMax=[]  DOutMin=[]  DOutMax=[]  NOutMin=[]  NOutMax=[]  SumOutMin=[]  SumOutMax=[]  SaturationOutMin=[]  SaturationOutMax=[]  PParamMin=[]  PParamMax=[]  IParamMin=[]  IParamMax=[]  DParamMin=[]  DParamMax=[]  NParamMin=[]  NParamMax=[]  KbParamMin=[]  KbParamMax=[]  KtParamMin=[]  KtParamMax=[]  KbOutMin=[]  KbOutMax=[]  KtOutMin=[]  KtOutMax=[]  IntegratorOutMin=[]  IntegratorOutMax=[]  FilterOutMin=[]  FilterOutMax=[]  SumI1OutMin=[]  SumI1OutMax=[]  SumI2OutMin=[]  SumI2OutMax=[]  SumI3OutMin=[]  SumI3OutMax=[]  SumI4OutMin=[]  SumI4OutMax=[]  SumDOutMin=[]  SumDOutMax=[]  DifferentiatorOutMin=[]  DifferentiatorOutMax=[]  FilterDiffOutCoefMin=[]  FilterDiffOutCoefMax=[]  ReciprocalOutMin=[]  ReciprocalOutMax=[]  SumDenOutMin=[]  SumDenOutMax=[]  SumNumOutMin=[]  SumNumOutMax=[]  DivideOutMin=[]  DivideOutMax=[]  UdiffTsProdOutMin=[]  UdiffTsProdOutMax=[]  NTsProdOutMin=[]  NTsProdOutMax=[]  UintegralTsProdOutMin=[]  UintegralTsProdOutMax=[]  UngainTsProdOutMin=[]  UngainTsProdOutMax=[]  ClampingZeroOutDataTypeStr=Inherit: Inherit via back propagation  ClampingZeroOutMin=[]  ClampingZeroOutMax=[]  FilterDenConstantOutDataTypeStr=Inherit: Inherit via back propagation  FilterDenConstantOutMin=[]  FilterDenConstantOutMax=[]  PCopyOutDataTypeStr=Inherit: Inherit via back propagation  PCopyOutMin=[]  PCopyOutMax=[]  NCopyOutDataTypeStr=Inherit: Inherit via back propagation  NCopyOutMin=[]  NCopyOutMax=[]  IntegratorContinuousStateAttributes=''  IntegratorStateMustResolveToSignalObject=off  IntegratorRTWStateStorageClass=Auto  FilterContinuousStateAttributes=''  FilterStateMustResolveToSignalObject=off  FilterRTWStateStorageClass=Auto  ParallelPVariant=InternalParameters  IdealPVariant=Disabled  IVariant=InternalParameters  DVariant=InternalParameters  IntegratorVariant=Continuous  SatVariant=Disabled  AWVariant=Passthrough  PCopyVariant=Disabled  TRVariant=Disabled  FdbkBlocksVariant=Forward  IdealPFdbkVariant=Disabled  SatFdbkVariant=Disabled  DerivativeFilterVariant=ContFilter  NVariant=InternalParameters  NCopyVariant=Disabled  FilterICVariant=InternalICsFilter  IntegratorICVariant=InternalICs  ExternalResetVariant=Disabled  TRSumVariant=Passthrough  SumFdbkVariant=Disabled  SumVariant=Sum_PID  TsampFilterVariant=InternalTs  TsampNgainVariant=Passthrough  TsampIntegralVariant=Disabled_SignalSpec  ExternalSaturationOutDataTypeStr=Inherit: Same as second input  DerivativeSourceVariant=ErrorSignal  PreIntVariant=InternalPreInt
  Pilot : Subsystem
  Pilot Joystick : aerolibanimutils/Pilot Joystick  JoystickID=Joystick1  OutputConfiguration=FourAxis  SampleTime=1/30
  Saturation : Saturate  UpperLimit=1  LowerLimit=0
  Saturation{1..3,5..6} (5 alike) : Saturate  UpperLimit=1  LowerLimit=-1
  Saturation4 : Saturate  UpperLimit=1  LowerLimit=0
  Saturation7 : Saturate  UpperLimit=40*pi/180  LowerLimit=-40*pi/180
  Scope : Scope  NumInputPorts=2
  Scope1 : Scope  NumInputPorts=2
  Scope{2..3,5..8} (6 alike) : Scope
  Scope4 : Scope  NumInputPorts=4
  Sqrt : Sqrt
  Subsystem1 : Subsystem
  Sum{,1..4} (5 alike) : Sum  Inputs=|++
  Sum5 : Sum  Inputs=|+-
  Sum6 : Sum  Inputs=|+-
  Sum7 : Sum  Inputs=|++-
  Zero-Order Hold : ZeroOrderHold  SampleTime=-1
  Zero-Order Hold1 : ZeroOrderHold  SampleTime=-1
  wires:
  Pilot/1(Pilot) -> De Havilland Beaver Airframe/2(Pilot)
  Environment/1(EnvBus) -> De Havilland Beaver Airframe/1(EnvirBus)
  Motion Conversion for Animation/1(FGInterface) -> FlightGear Preconfigured 6DoF Animation/1
  Sum/1 -> Scope4/3, Saturation4/1  "T"
  Sum2/1 -> Scope4/2, Saturation3/1  "elevator"
  Subsystem1/1(T) -> Zero-Order Hold/1
  Subsystem1/2(Elev) -> Zero-Order Hold1/1
  Constant/1 -> Scope/1, Subsystem1/1(Exp_High)
  Bus Selector/4 -> Subsystem1/6(Abe_tot)  "<Abe_tot>"
  Bus Selector/3 -> Scope/2, Subsystem1/5(High)  "<H>"
  Bus Selector/2 -> Scope1/2, Subsystem1/4(Ve_tot)  "<Ve_tot>"
  Bus Selector/1 -> Subsystem1/3(TAngle)  "<TAngle>"
  Constant1/1 -> Scope1/1, Subsystem1/2(Exp_Speed)
  Zero-Order Hold/1 -> Saturation/1
  Zero-Order Hold1/1 -> Saturation1/1
  Saturation/1 -> Scope2/1, [T_ctl]
  Saturation1/1 -> Scope3/1, [E_ctl]
  Saturation2/1 -> Pilot/1(In1)
  Saturation3/1 -> Pilot/2(In2)
  Saturation4/1 -> Pilot/3(In3)
  Saturation5/1 -> Pilot/4(In4)
  Sum1/1 -> Scope4/1, Saturation2/1
  elevator/1 -> Sum2/1
  T/1 -> Sum/1
  Sum3/1 -> Scope4/4, Saturation5/1
  Bus Selector1/2 -> Scope6/1  "<xyh>"
  Bus Selector1/1 -> Scope5/1  "<Ve>"
  Bus Selector1/3 -> Angle Conversion5/1  "<phi_theta_psi>"
  Pilot Joystick/4 -> Sum4/1
  Constant2/1 -> Sum4/2
  De Havilland Beaver Airframe/1(ACBus) -> Bus Selector2/1, Bus Selector1/1, Environment/1(ACBus), Bus Selector/1, Motion Conversion for Animation/1(ACBus)
  Bus Selector2/3 -> Demux1/1  "<phi_theta_psi>"
  Bus Selector2/2 -> Demux/1  "<xyh>"
  Bus Selector2/1 -> Dot Product/1, Dot Product/2  "<Ve>"
  Dot Product/1 -> Sqrt/1
  Sqrt/1 -> [V]  "V"
  Demux/3 -> [H]  "h"
  Demux1/2 -> Angle Conversion1/1  "theta"
  [V] -> Sum5/2
  Constant3/1 -> Sum5/1
  Sum5/1 -> PID Controller/1
  [H] -> Sum6/2
  Constant4/1 -> Sum6/1
  Saturation7/1 -> Sum7/1
  [theta] -> Sum7/3
  Sum7/1 -> Scope8/1, PID Controller1/1
  Sum6/1 -> PID Controller2/1
  PID Controller1/1 -> Saturation6/1
  Constant5/1 -> Sum7/2
  Constant6/1 -> Saturation7/1
  Angle Conversion5/1 -> Scope7/1
  Angle Conversion1/1 -> [theta]

== system asbdhc2(1)/De Havilland Beaver Airframe ==
  EnvirBus : Inport
  Pilot : Inport  Port=2
  Aircraft Dynamics : Subsystem
  Calculate Parameters : Subsystem
  ACBus : Outport  VectorParamsAs1DForOutWhenUnconnected=off
  wires:
  Pilot/1 -> Aircraft Dynamics/1(Pilot)
  Aircraft Dynamics/1(AC Bus) -> ACBus/1, Calculate Parameters/2(ACBus)
  EnvirBus/1 -> Aircraft Dynamics/2(EnvirBus), Calculate Parameters/1(EnvirBus)
  Calculate Parameters/1(FltParams) -> Aircraft Dynamics/3(FltParams)

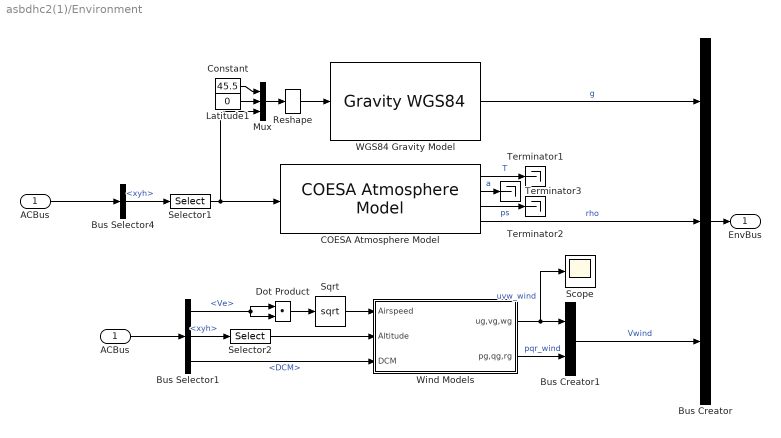
== system asbdhc2(1)/Environment ==
  ACBus : Inport
  "ACBus " : InportShadow
  Bus Creator : BusCreator  Inputs=3
  Bus Creator1 : BusCreator  Inputs=2
  Bus Selector1 : BusSelector  OutputSignals=Ve,xyh,DCM
  Bus Selector4 : BusSelector  OutputSignals=xyh
  COESA Atmosphere Model : aerolibatmos2/COESA Atmosphere Model  units=Metric (MKS)  spec=1976 COESA-extended U.S. Standard Atmosphere  model=Profile  profile_var=High temperature  profile_percent=1%  profile_alt=5 km (16404 ft)  envelope_var=High temperature  envelope_percent=1%  action=Warning
  Constant : Constant  Value=45.5
  Dot Product : DotProduct  OutDataTypeStr=Inherit: Inherit via internal rule
  Latitude1 : Constant  Value=0
  Mux : Mux  Inputs=3
  Reshape : Reshape  OutputDimensionality=Row vector (2-D)
  Scope : Scope
  Selector1 : Selector  IndexMode=Zero-based  InputPortWidth=3  IndexOptions=Index vector (dialog)  Indices=2  OutputSizes=1
  Selector2 : Selector  IndexMode=Zero-based  InputPortWidth=3  IndexOptions=Index vector (dialog)  Indices=2  OutputSizes=1
  Sqrt : Sqrt
  Terminator1 : Terminator
  Terminator2 : Terminator
  Terminator3 : Terminator
  "WGS84 Gravity Model  " : GravityWGS84  action=None
  Wind Models : Subsystem
  EnvBus : Outport  VectorParamsAs1DForOutWhenUnconnected=off
  wires:
  COESA Atmosphere Model/4 -> Bus Creator/2  "rho"
  COESA Atmosphere Model/1 -> Terminator1/1  "T"
  COESA Atmosphere Model/3 -> Terminator2/1  "ps"
  COESA Atmosphere Model/2 -> Terminator3/1  "a"
  Selector1/1 -> COESA Atmosphere Model/1, Mux/3
  Bus Selector1/3 -> Wind Models/3(DCM)  "<DCM>"
  Wind Models/2(pg,qg,rg) -> Bus Creator1/2  "pqr_wind"
  Wind Models/1(ug,vg,wg) -> Scope/1, Bus Creator1/1  "uvw_wind"
  Bus Creator1/1 -> Bus Creator/3  "Vwind"
  Dot Product/1 -> Sqrt/1
  Sqrt/1 -> Wind Models/1(Airspeed)
  Bus Creator/1 -> EnvBus/1
  ACBus/1 -> Bus Selector4/1
  Bus Selector4/1 -> Selector1/1  "<xyh>"
  "ACBus "/1 -> Bus Selector1/1
  Bus Selector1/2 -> Selector2/1  "<xyh>"
  Selector2/1 -> Wind Models/2(Altitude)
  Bus Selector1/1 -> Dot Product/1, Dot Product/2  "<Ve>"
  Constant/1 -> Mux/1
  Latitude1/1 -> Mux/2
  Mux/1 -> Reshape/1
  "WGS84 Gravity Model  "/1 -> Bus Creator/1  "g"
  Reshape/1 -> "WGS84 Gravity Model  "/1

== system asbdhc2(1)/Motion Conversion for Animation ==
  ACBus : Inport
  Bus Selector : BusSelector  OutputSignals=phi_theta_psi
  Bus Selector1 : BusSelector  OutputSignals=Xe  OutputAsBus=on
  Constant : Constant  Value=0
  Flat Earth to LLA : aerolibtransform2/Flat Earth to LLA  units=Metric (MKS)  ptype=Earth (WGS84)  F=1/298.257223563  R=6378137  refPosPort=off  LL0=[37.6272 -122.3896]  psi=0
  Mux : Mux  Inputs=2
  Mux1 : Mux  Inputs=2
  Selector : Selector  IndexMode=Zero-based  InputPortWidth=2  IndexOptions=Index vector (dialog)  Indices=[1 0]  OutputSizes=1
  FGInterface : Outport  VectorParamsAs1DForOutWhenUnconnected=off
  wires:
  Mux1/1 -> FGInterface/1
  Constant/1 -> Flat Earth to LLA/2
  Bus Selector/1 -> Mux1/2  "<phi_theta_psi>"
  Mux/1 -> Mux1/1
  Flat Earth to LLA/2 -> Mux/2
  Flat Earth to LLA/1 -> Selector/1
  Bus Selector1/1 -> Flat Earth to LLA/1
  ACBus/1 -> Bus Selector/1, Bus Selector1/1
  Selector/1 -> Mux/1

== system asbdhc2(1)/Pilot ==
  In1 : Inport
  In2 : Inport  Port=2
  In3 : Inport  Port=3
  In4 : Inport  Port=4
  Bus Creator : BusCreator  Inputs=2
  Flap : Constant  Value=0
  Input Signal Conditioning : Subsystem
  Mux2 : Mux  Inputs=3
  Pilot Joystick : aerolibanimutils/Pilot Joystick  Commented=on  JoystickID=None  OutputConfiguration=FourAxis  SampleTime=1/30
  Rate Transition1 : RateTransition  OutPortSampleTime=0
  Rate Transition2 : RateTransition  OutPortSampleTime=0
  Pilot : Outport  VectorParamsAs1DForOutWhenUnconnected=off
  wires:
  Flap/1 -> Input Signal Conditioning/3(Flap)
  Rate Transition1/1 -> Input Signal Conditioning/1(Stick / Throt)
  Rate Transition2/1 -> Input Signal Conditioning/2(Rudder)
  Input Signal Conditioning/1(uaero) -> Bus Creator/1  "uaero"
  Input Signal Conditioning/2(uprop) -> Bus Creator/2  "uprop"
  Bus Creator/1 -> Pilot/1
  Mux2/1 -> Rate Transition1/1
  In1/1 -> Mux2/1
  In2/1 -> Mux2/2
  In3/1 -> Mux2/3
  In4/1 -> Rate Transition2/1

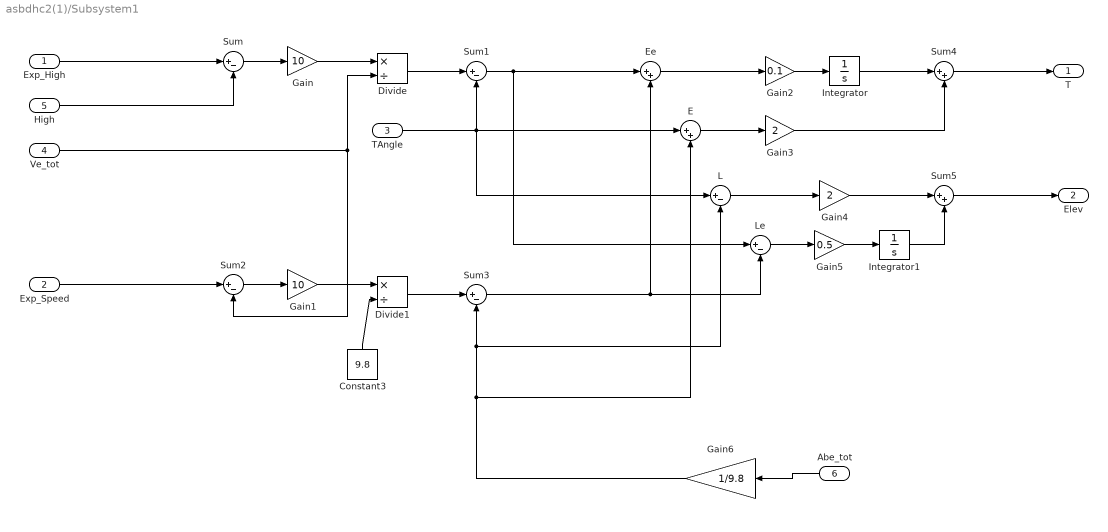
== system asbdhc2(1)/Subsystem1 ==
  Exp_High : Inport
  Exp_Speed : Inport  Port=2
  TAngle : Inport  Port=3
  Ve_tot : Inport  Port=4
  High : Inport  Port=5
  Abe_tot : Inport  Port=6
  Constant3 : Constant  Value=9.8
  Divide : Product  Inputs=*/
  Divide1 : Product  Inputs=*/
  E : Sum  Inputs=|++
  Ee : Sum  Inputs=|++
  Gain : Gain  Gain=10
  Gain1 : Gain  Gain=10
  Gain2 : Gain  Gain=0.1
  Gain3 : Gain  Gain=2
  Gain4 : Gain  Gain=2
  Gain5 : Gain  Gain=0.5
  Gain6 : Gain  Gain=1/9.8
  Integrator : Integrator
  Integrator1 : Integrator
  L : Sum  Inputs=|+-
  Le : Sum  Inputs=|+-
  Sum{,1..3} (4 alike) : Sum  Inputs=|+-
  Sum4 : Sum  Inputs=|++
  Sum5 : Sum  Inputs=|++
  T : Outport
  Elev : Outport  Port=2
  wires:
  Sum1/1 -> Le/1, Ee/1
  Exp_Speed/1 -> Sum2/1
  Sum/1 -> Gain/1
  Le/1 -> Gain5/1
  Constant3/1 -> Divide1/2
  Integrator1/1 -> Sum5/2
  Sum4/1 -> T/1
  Sum3/1 -> Le/2, Ee/2
  E/1 -> Gain3/1
  Gain6/1 -> Sum3/2, L/2, E/2
  Gain1/1 -> Divide1/1
  Exp_High/1 -> Sum/1
  Ve_tot/1 -> Divide/2, Sum2/2
  Gain3/1 -> Sum4/2
  Gain4/1 -> Sum5/1
  Abe_tot/1 -> Gain6/1
  Gain2/1 -> Integrator/1
  Ee/1 -> Gain2/1
  Sum2/1 -> Gain1/1
  Divide/1 -> Sum1/1
  Integrator/1 -> Sum4/1
  L/1 -> Gain4/1
  TAngle/1 -> L/1, E/1, Sum1/2
  Gain/1 -> Divide/1
  Sum5/1 -> Elev/1
  Gain5/1 -> Integrator1/1
  Divide1/1 -> Sum3/1
  High/1 -> Sum/2

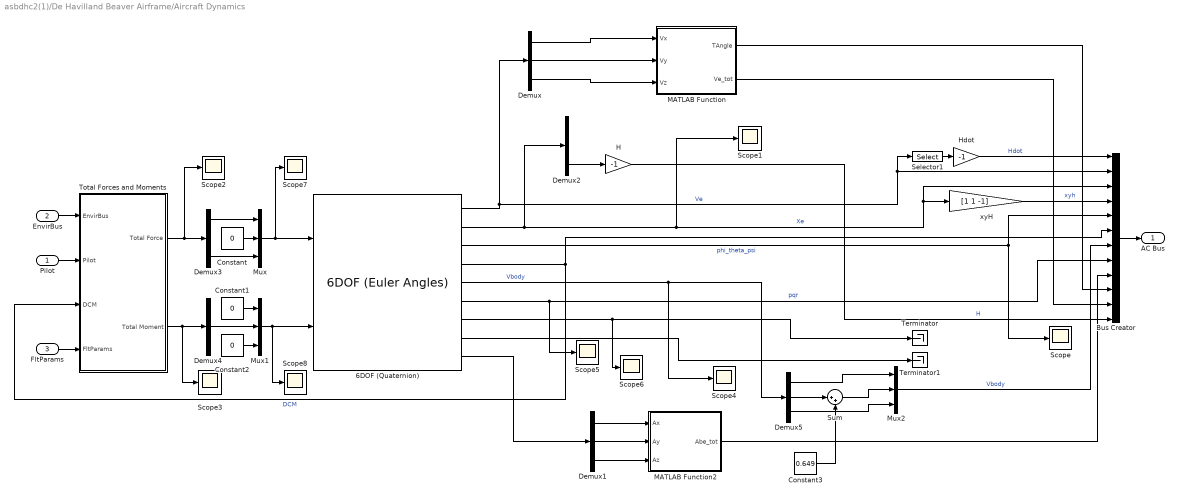
== system asbdhc2(1)/De Havilland Beaver Airframe/Aircraft Dynamics ==
  Pilot : Inport
  EnvirBus : Inport  Port=2
  FltParams : Inport  Port=3
  6DOF (Quaternion) : shared6dof/6DOF (Euler Angles)  units=Metric (MKS)  mtype=Fixed  rep=Euler Angles  xme_0=xme_0  Vm_0=[44.54 0 5.836]  eul_0=[beaver_init_roll, 0, 113/180*pi]  pm_0=[beaver_init_p, beaver_init_q, beaver_init_r]  mass_0=2000  mass_e=0  mass_f=0  inertia="[5.787969e3  0 1.1764e2; 0 6.92893e3 0; -1.1764e2 0 1.1578329e4]"  inertia_e=eye(3)  inertia_f=eye(3)  k_quat=1.0  vre_flag=on  abi_flag=on  aMode=aMode  xme_statename=''  Vm_statename=''  eul_statename=''  quat_statename=''  pm_statename=''  mass_statename=''
  Bus Creator : BusCreator  Inputs=12
  Constant : Constant  Value=0
  Constant1 : Constant  Value=0
  Constant2 : Constant  Value=0
  Constant3 : Constant  Value=0.649
  Demux{,1..5} (6 alike) : Demux  Outputs=3
  H : Gain  Gain=-1  SaturateOnIntegerOverflow=on  OutDataTypeStr=Inherit: Same as input  ParamDataTypeStr=Inherit: Same as input
  Hdot : Gain  Gain=-1  SaturateOnIntegerOverflow=on  OutDataTypeStr=Inherit: Same as input  ParamDataTypeStr=Inherit: Same as input
  MATLAB Function : MATLAB Function  TreatAsAtomicUnit=on
  MATLAB Function2 : MATLAB Function  TreatAsAtomicUnit=on
  Mux : Mux  Inputs=3
  Mux1 : Mux  Inputs=3
  Mux2 : Mux  Inputs=3
  Scope{,1..8} (9 alike) : Scope
  Selector1 : Selector  IndexMode=Zero-based  InputPortWidth=3  IndexOptions=Index vector (dialog)  Indices=2  OutputSizes=1
  Sum : Sum  Inputs=|++
  Terminator : Terminator
  Terminator1 : Terminator
  Total Forces and Moments : Subsystem
  xyH : Gain  Gain=[1 1 -1]  SaturateOnIntegerOverflow=on  OutDataTypeStr=Inherit: Same as input  ParamDataTypeStr=Inherit: Same as input
  AC Bus : Outport  VectorParamsAs1DForOutWhenUnconnected=off
  wires:
  6DOF (Quaternion)/4 -> Total Forces and Moments/3(DCM), Bus Creator/6  "DCM"
  6DOF (Quaternion)/3 -> Scope/1, Bus Creator/5  "phi_theta_psi"
  6DOF (Quaternion)/2 -> Demux2/1, Scope1/1, xyH/1, Bus Creator/3  "Xe"
  6DOF (Quaternion)/5 -> Scope4/1, Demux5/1  "Vbody"
  6DOF (Quaternion)/7 -> Scope6/1, Terminator/1
  6DOF (Quaternion)/1 -> Demux/1, Selector1/1, Bus Creator/2  "Ve"
  Pilot/1 -> Total Forces and Moments/2(Pilot)
  Selector1/1 -> Hdot/1
  xyH/1 -> Bus Creator/4  "xyh"
  Hdot/1 -> Bus Creator/1  "Hdot"
  6DOF (Quaternion)/8 -> Terminator1/1
  Bus Creator/1 -> AC Bus/1
  EnvirBus/1 -> Total Forces and Moments/1(EnvirBus)
  6DOF (Quaternion)/6 -> Scope5/1, Bus Creator/8  "pqr"
  FltParams/1 -> Total Forces and Moments/4(FltParams)
  Demux/2 -> MATLAB Function/2(Vy)
  Demux/1 -> MATLAB Function/1(Vx)
  Demux/3 -> MATLAB Function/3(Vz)
  Demux1/1 -> MATLAB Function2/1(Ax)
  Demux1/2 -> MATLAB Function2/2(Ay)
  Demux1/3 -> MATLAB Function2/3(Az)
  6DOF (Quaternion)/9 -> Demux1/1
  MATLAB Function2/1(Abe_tot) -> Bus Creator/9
  MATLAB Function/1(TAngle) -> Bus Creator/10
  MATLAB Function/2(Ve_tot) -> Bus Creator/11
  Demux2/3 -> H/1
  H/1 -> Bus Creator/12  "H"
  Constant/1 -> Mux/2
  Demux3/1 -> Mux/1
  Demux3/3 -> Mux/3
  Total Forces and Moments/1(Total Force) -> Scope2/1, Demux3/1
  Mux/1 -> Scope7/1, 6DOF (Quaternion)/1
  Total Forces and Moments/2(Total Moment) -> Scope3/1, Demux4/1
  Mux1/1 -> Scope8/1, 6DOF (Quaternion)/2
  Constant1/1 -> Mux1/1
  Constant2/1 -> Mux1/3
  Demux4/2 -> Mux1/2
  Demux5/2 -> Sum/1
  Constant3/1 -> Sum/2
  Demux5/1 -> Mux2/1
  Sum/1 -> Mux2/2
  Demux5/3 -> Mux2/3
  Mux2/1 -> Bus Creator/7  "Vbody"

== system asbdhc2(1)/De Havilland Beaver Airframe/Calculate Parameters ==
  EnvirBus : Inport
  ACBus : Inport  Port=2
  "ACBus " : InportShadow  Port=2
  Bus Creator : BusCreator  Inputs=5
  Bus Selector1 : BusSelector  OutputSignals=rho
  Bus Selector2 : BusSelector  OutputSignals=Vbody
  Bus Selector3 : BusSelector  OutputSignals=pqr,Ve
  Bus Selector4 : BusSelector  OutputSignals=Vwind.uvw_wind,Vwind.pqr_wind
  Dynamic Pressure : aerolibasang/Dynamic Pressure
  "Incidence, Sideslip, & Airspeed" : aerolibasang/Incidence, Sideslip, & Airspeed
  Scope : Scope
  Sum2 : Sum  Inputs=|++  InputSameDT=on  SaturateOnIntegerOverflow=on  OutDataTypeStr=Inherit: Same as first input
  Sum4 : Sum  Inputs=+-|  InputSameDT=on  SaturateOnIntegerOverflow=on  OutDataTypeStr=Inherit: Same as first input
  FltParams : Outport  VectorParamsAs1DForOutWhenUnconnected=off
  wires:
  "ACBus "/1 -> Bus Selector2/1
  Bus Creator/1 -> FltParams/1
  Bus Selector3/1 -> Sum2/2  "<pqr>"
  ACBus/1 -> Bus Selector3/1
  Bus Selector1/1 -> Dynamic Pressure/2  "<rho>"
  EnvirBus/1 -> Bus Selector1/1, Bus Selector4/1
  Dynamic Pressure/1 -> Bus Creator/5  "Qdyn"
  Bus Selector3/2 -> Dynamic Pressure/1  "<Ve>"
  Bus Selector4/2 -> Sum2/1  "<pqr_wind>"
  Sum4/1 -> "Incidence, Sideslip, & Airspeed"/1
  "Incidence, Sideslip, & Airspeed"/1 -> Bus Creator/1  "alpha"
  "Incidence, Sideslip, & Airspeed"/2 -> Bus Creator/2  "beta"
  "Incidence, Sideslip, & Airspeed"/3 -> Bus Creator/3  "V"
  Bus Selector2/1 -> Scope/1, Sum4/1  "<Vbody>"
  Bus Selector4/1 -> Sum4/2  "<uvw_wind>"
  Sum2/1 -> Bus Creator/4  "pqr_tot"

== system asbdhc2(1)/Environment/Wind Models ==
  Airspeed : Inport  Unit=m/s
  Altitude : Inport  Port=2  Unit=meter
  DCM : Inport  Port=3
  "DCM " : InportShadow  Port=3
  Discrete Wind Gust Model : aerolibwind2/Discrete Wind Gust Model  units=Metric (MKS)  Gx=off  Gy=off  Gz=off  t_0=20  d_m=[120 120 80]  v_m=[3.5 3.5 3.0]
  Dryden Wind Turbulence Model (Continuous (+q -r)) : aerolibwind2/Dryden Wind Turbulence Model  (Continuous (+q -r))  units=Metric (MKS)  spec=MIL-F-8785C  model=Continuous Dryden (+q -r)  W20=5  Wdeg=0  TurbProb=10^-2 - Light  L_high=533.4  Wingspan=4  ts=0.1  Seed=[23341 23342 23343 23344]  T_on=off
  Sum : Sum  Inputs=+++  InputSameDT=on  SaturateOnIntegerOverflow=on  OutDataTypeStr=Inherit: Same as first input
  Wind Shear Model : aerolibwind2/Wind Shear Model  units=Metric (MKS)  phase=Category C - Terminal Flight Phase  W_20=0  Wdeg=0
  ug,vg,wg : Outport  Unit=m/s  VectorParamsAs1DForOutWhenUnconnected=off
  pg,qg,rg : Outport  Port=2  Unit=rad/second  VectorParamsAs1DForOutWhenUnconnected=off
  wires:
  "DCM "/1 -> Dryden Wind Turbulence Model (Continuous (+q -r))/3
  Wind Shear Model/1 -> Sum/1
  Dryden Wind Turbulence Model (Continuous (+q -r))/1 -> Sum/2
  Discrete Wind Gust Model/1 -> Sum/3
  Sum/1 -> ug,vg,wg/1
  DCM/1 -> Wind Shear Model/2
  Airspeed/1 -> Dryden Wind Turbulence Model (Continuous (+q -r))/2, Discrete Wind Gust Model/1
  Dryden Wind Turbulence Model (Continuous (+q -r))/2 -> pg,qg,rg/1
  Altitude/1 -> Dryden Wind Turbulence Model (Continuous (+q -r))/1, Wind Shear Model/1

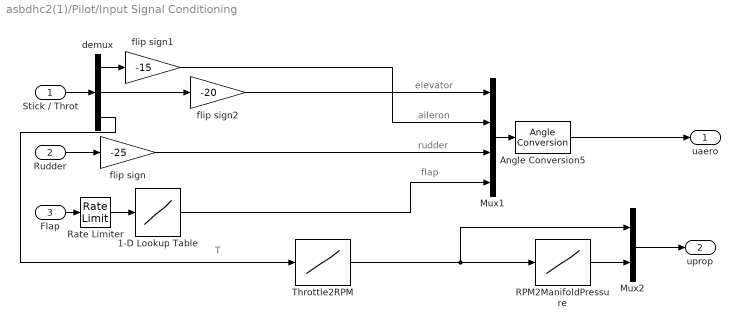
== system asbdhc2(1)/Pilot/Input Signal Conditioning ==
  note: flap
  note: rudder
  note: T
  note: elevator
  note: aileron
  Stick / Throt : Inport
  Rudder : Inport  Port=2
  Flap : Inport  Port=3
  1-D Lookup Table : Lookup_n-D  NumberOfTableDimensions=1  LookupTableObject=''  BreakpointsForDimension1=[0:3]  Table=[0 4 10 20]  SaturateOnIntegerOverflow=on
  Angle Conversion5 : aerolibconvert2/Angle Conversion  IU=deg  OU=rad
  Mux1 : Mux
  Mux2 : Mux  Inputs=2
  RPM2ManifoldPressure : Lookup_n-D  NumberOfTableDimensions=1  LookupTableObject=''  BreakpointsForDimension1=[0 1800 2300]  IndexSearchMethod=Linear search  BeginIndexSearchUsingPreviousIndexResult=on  Table=[0 22.5735 26]  ExtrapMethod=Clip
  Rate Limiter : RateLimiter  RisingSlewLimit=0.5  FallingSlewLimit=-0.5
  Throttle2RPM : Lookup_n-D  NumberOfTableDimensions=1  LookupTableObject=''  BreakpointsForDimension1=(1/6)*(3+([-3:3]))  IndexSearchMethod=Linear search  BeginIndexSearchUsingPreviousIndexResult=on  Table=((1+tanh([-3:3]))/(1+tanh(2.65))-0.0025)*2300  ExtrapMethod=Clip
  demux : Demux  Outputs=3
      settings: DisplayOption=none
  flip sign : Gain  Gain=-25  SaturateOnIntegerOverflow=on  OutDataTypeStr=Inherit: Same as input  ParamDataTypeStr=Inherit: Same as input
  flip sign1 : Gain  Gain=-15  SaturateOnIntegerOverflow=on  OutDataTypeStr=Inherit: Same as input  ParamDataTypeStr=Inherit: Same as input
  flip sign2 : Gain  Gain=-20  SaturateOnIntegerOverflow=on  OutDataTypeStr=Inherit: Same as input  ParamDataTypeStr=Inherit: Same as input
  uaero : Outport  Unit=rad  VectorParamsAs1DForOutWhenUnconnected=off
  uprop : Outport  Port=2  VectorParamsAs1DForOutWhenUnconnected=off
  wires:
  demux/3 -> Throttle2RPM/1
  Flap/1 -> Rate Limiter/1
  Rate Limiter/1 -> 1-D Lookup Table/1
  Stick / Throt/1 -> demux/1
  Rudder/1 -> flip sign/1
  1-D Lookup Table/1 -> Mux1/4
  demux/1 -> flip sign1/1
  demux/2 -> flip sign2/1
  Mux1/1 -> Angle Conversion5/1
  Angle Conversion5/1 -> uaero/1
  RPM2ManifoldPressure/1 -> Mux2/2
  Mux2/1 -> uprop/1
  flip sign/1 -> Mux1/3
  Throttle2RPM/1 -> Mux2/1, RPM2ManifoldPressure/1
  flip sign1/1 -> Mux1/2
  flip sign2/1 -> Mux1/1

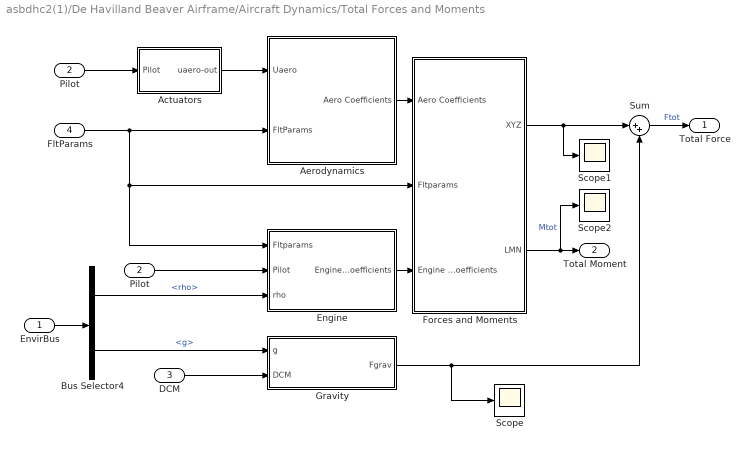
== system asbdhc2(1)/De Havilland Beaver Airframe/Aircraft Dynamics/Total Forces and Moments ==
  EnvirBus : Inport
  Pilot : Inport  Port=2
  DCM : Inport  Port=3
  FltParams : Inport  Port=4
  Actuators : Subsystem
  Aerodynamics : Subsystem
  Bus Selector4 : BusSelector  OutputSignals=rho,g
  "Engine " : Subsystem
  Forces and Moments : Subsystem
  "Gravity " : Subsystem
  "Pilot " : InportShadow  Port=2
  Scope : Scope
  Scope1 : Scope
  Scope2 : Scope
  Sum : Sum  Inputs=|++  InputSameDT=on  SaturateOnIntegerOverflow=on  OutDataTypeStr=Inherit: Same as first input
  Total Force : Outport  Unit=N  VectorParamsAs1DForOutWhenUnconnected=off
  Total Moment : Outport  Port=2  Unit=N*m  VectorParamsAs1DForOutWhenUnconnected=off
  wires:
  Forces and Moments/1(XYZ) -> Scope1/1, Sum/1
  "Engine "/1(Engine Coefficients) -> Forces and Moments/3(Engine Coefficients)
  "Gravity "/1(Fgrav) -> Scope/1, Sum/2
  Aerodynamics/1(Aero Coefficients) -> Forces and Moments/1(Aero Coefficients)
  Pilot/1 -> Actuators/1(Pilot)
  Bus Selector4/1 -> "Engine "/3(rho)  "<rho>"
  DCM/1 -> "Gravity "/2(DCM)
  Bus Selector4/2 -> "Gravity "/1(g)  "<g>"
  Sum/1 -> Total Force/1  "Ftot"
  Forces and Moments/2(LMN) -> Scope2/1, Total Moment/1  "Mtot"
  "Pilot "/1 -> "Engine "/2(Pilot)
  FltParams/1 -> Forces and Moments/2(Fltparams), "Engine "/1(Fltparams), Aerodynamics/2(FltParams)
  Actuators/1(uaero-out) -> Aerodynamics/1(Uaero)
  EnvirBus/1 -> Bus Selector4/1

== system asbdhc2(1)/De Havilland Beaver Airframe/Aircraft Dynamics/Total Forces and Moments/Actuators ==
  Pilot : Inport
  Bus Selector2 : BusSelector  OutputSignals=uaero
  Demux : Demux
  Initial inputs for aero : Constant  Commented=on  Value=uaero0
  Mux : Mux
  Sum1 : Sum  Inputs=++|  InputSameDT=on  SaturateOnIntegerOverflow=on  OutDataTypeStr=Inherit: Same as first input
  uaero-out : Outport  Unit=rad  VectorParamsAs1DForOutWhenUnconnected=off
  wires:
  Pilot/1 -> Bus Selector2/1
  Initial inputs for aero/1 -> Sum1/1
  Sum1/1 -> uaero-out/1
  Bus Selector2/1 -> Demux/1  "<uaero>"
  Demux/4 -> Mux/4
  Demux/1 -> Mux/1
  Demux/2 -> Mux/2
  Demux/3 -> Mux/3
  Mux/1 -> Sum1/2

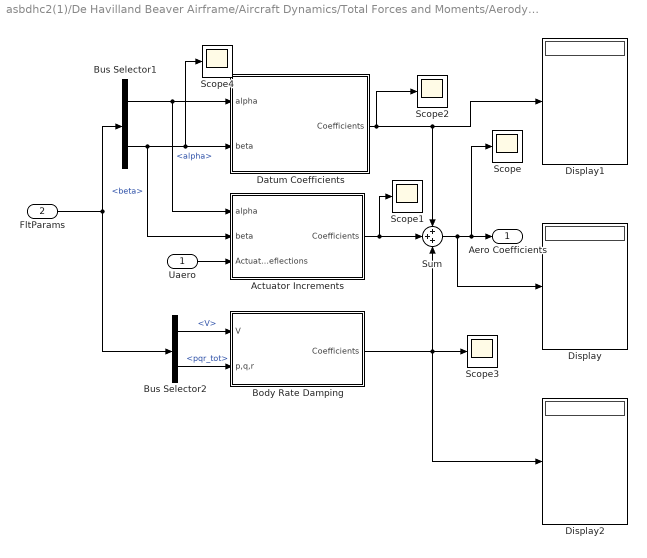
== system asbdhc2(1)/De Havilland Beaver Airframe/Aircraft Dynamics/Total Forces and Moments/Aerodynamics ==
  Uaero : Inport  Unit=rad
  FltParams : Inport  Port=2
  Actuator Increments : Subsystem
  Body Rate Damping : Subsystem
  Bus Selector1 : BusSelector  OutputSignals=alpha,beta
  Bus Selector2 : BusSelector  OutputSignals=V,pqr_tot
  Datum Coefficients : Subsystem
  Display : Display
  Display1 : Display
  Display2 : Display
  Scope{,1..4} (5 alike) : Scope
  Sum : Sum  Inputs=+++  SaturateOnIntegerOverflow=on
  Aero Coefficients : Outport  VectorParamsAs1DForOutWhenUnconnected=off
  wires:
  Bus Selector1/2 -> Actuator Increments/2(beta), Scope4/1, Datum Coefficients/2(beta)  "<beta>"
  Sum/1 -> Scope/1, Aero Coefficients/1, Display/1
  Body Rate Damping/1(Coefficients) -> Display2/1, Scope3/1, Sum/3
  Datum Coefficients/1(Coefficients) -> Scope2/1, Sum/1, Display1/1
  Actuator Increments/1(Coefficients) -> Scope1/1, Sum/2
  Bus Selector2/1 -> Body Rate Damping/1(V)  "<V>"
  Bus Selector2/2 -> Body Rate Damping/2(p,q,r)  "<pqr_tot>"
  Uaero/1 -> Actuator Increments/3(Actuator Deflections)
  Bus Selector1/1 -> Actuator Increments/1(alpha), Datum Coefficients/1(alpha)  "<alpha>"
  FltParams/1 -> Bus Selector1/1, Bus Selector2/1

== system asbdhc2(1)/De Havilland Beaver Airframe/Aircraft Dynamics/Total Forces and Moments/Engine  ==
  Fltparams : Inport
  Pilot : Inport  Port=2
  rho : Inport  Port=3  Unit=kg/m^3
  Bus Selector4 : BusSelector  OutputSignals=V,alpha
  Display : Display
  Scope : Scope
  eng : Subsystem
  pow : Subsystem
  Engine Coefficients : Outport  VectorParamsAs1DForOutWhenUnconnected=off
  wires:
  Bus Selector4/1 -> pow/3(V)  "<V>"
  rho/1 -> pow/1(rho)
  Bus Selector4/2 -> eng/2(alpha)  "<alpha>"
  eng/1(Cprop) -> Engine Coefficients/1, Scope/1, Display/1
  Pilot/1 -> pow/2(Pilot)
  pow/1(dpt) -> eng/1(dpt)
  Fltparams/1 -> Bus Selector4/1

== system asbdhc2(1)/De Havilland Beaver Airframe/Aircraft Dynamics/Total Forces and Moments/Forces and Moments ==
  Aero Coefficients : Inport
  Fltparams : Inport  Port=2
  Engine Coefficients : Inport  Port=3
  Aerodynamic Forces and Moments : aerolibadyn/Aerodynamic Forces and Moments   inputAxes=Body  outputForceAxes=Body  outputMomentAxes=Body  S=beaver_S  b=beaver_b  cbar=beaver_c
  Bus Selector4 : BusSelector  OutputSignals=Qdyn
  Display : Display
  Display1 : Display
  Display2 : Display
  Scope : Scope
  Sum : Sum  Inputs=++|  InputSameDT=on  SaturateOnIntegerOverflow=on  OutDataTypeStr=Inherit: Same as first input
  neglect center of gravity and center of pressure effects : Constant  Value=[0 0 0]
  XYZ : Outport  Unit=N  VectorParamsAs1DForOutWhenUnconnected=off
  LMN : Outport  Port=2  Unit=N*m  VectorParamsAs1DForOutWhenUnconnected=off
  wires:
  Sum/1 -> Display1/1, Aerodynamic Forces and Moments/1
  Aero Coefficients/1 -> Display2/1, Sum/2
  Engine Coefficients/1 -> Sum/1, Display/1
  Aerodynamic Forces and Moments/2 -> Scope/1, LMN/1
  Fltparams/1 -> Bus Selector4/1
  Aerodynamic Forces and Moments/1 -> XYZ/1
  neglect center of gravity and center of pressure effects/1 -> Aerodynamic Forces and Moments/3, Aerodynamic Forces and Moments/4
  Bus Selector4/1 -> Aerodynamic Forces and Moments/2  "<Qdyn>"

== system asbdhc2(1)/De Havilland Beaver Airframe/Aircraft Dynamics/Total Forces and Moments/Gravity  ==
  g : Inport  Unit=m/s^2
  DCM : Inport  Port=2
  Gravity in Earth Axes : Gain  Gain=beaver_mass  SaturateOnIntegerOverflow=on  OutDataTypeStr=Inherit: Same as input  ParamDataTypeStr=Inherit: Same as input
  Inertial to Body : Product  Multiplication=Matrix(*)  InputSameDT=on  SaturateOnIntegerOverflow=on  OutDataTypeStr=Inherit: Same as first input
  Reshape : Reshape  OutputDimensionality=Column vector (2-D)
  Reshape1 : Reshape
  Fgrav : Outport  Unit=N  VectorParamsAs1DForOutWhenUnconnected=off
  wires:
  Inertial to Body/1 -> Reshape1/1
  g/1 -> Gravity in Earth Axes/1
  DCM/1 -> Inertial to Body/1
  Gravity in Earth Axes/1 -> Reshape/1
  Reshape/1 -> Inertial to Body/2
  Reshape1/1 -> Fgrav/1

== system asbdhc2(1)/De Havilland Beaver Airframe/Aircraft Dynamics/Total Forces and Moments/Aerodynamics/Actuator Increments ==
  alpha : Inport  Unit=rad
  beta : Inport  Port=2  Unit=rad
  Actuator Deflections : Inport  Port=3  Unit=rad
  Aileron : Subsystem
  Display : Display
  Elevator : Subsystem
  Flap : Subsystem
  Rudder : Subsystem
  Sum : Sum  Inputs=++++  InputSameDT=on  SaturateOnIntegerOverflow=on  OutDataTypeStr=Inherit: Same as first input
  Coefficients : Outport  VectorParamsAs1DForOutWhenUnconnected=off
  wires:
  Actuator Deflections/1 -> Flap/2(Actuators), Aileron/2(Actuators), Elevator/1(Actuators), Rudder/2(Actuators)
  alpha/1 -> Flap/1(Alpha), Rudder/1(Alpha), Aileron/1(alpha)
  beta/1 -> Elevator/2(Beta)
  Aileron/1(delCoeff) -> Sum/1
  Elevator/1(delCoeff) -> Sum/2
  Rudder/1(delCoeff) -> Sum/3
  Flap/1(delCoeff) -> Sum/4
  Sum/1 -> Coefficients/1, Display/1

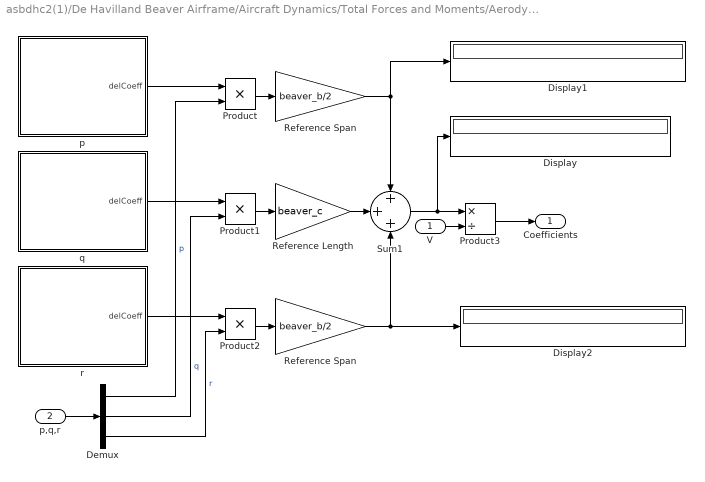
== system asbdhc2(1)/De Havilland Beaver Airframe/Aircraft Dynamics/Total Forces and Moments/Aerodynamics/Body Rate Damping ==
  V : Inport  Unit=m/second
  p,q,r : Inport  Port=2  Unit=rad/second
  Demux : Demux  Outputs=3
      settings: DisplayOption=none
  Display : Display
  Display1 : Display
  Display2 : Display
  Product : Product  InputSameDT=on  SaturateOnIntegerOverflow=on  OutDataTypeStr=Inherit: Same as first input
  Product1 : Product  InputSameDT=on  SaturateOnIntegerOverflow=on  OutDataTypeStr=Inherit: Same as first input
  Product2 : Product  InputSameDT=on  SaturateOnIntegerOverflow=on  OutDataTypeStr=Inherit: Same as first input
  Product3 : Product  Inputs=*/  InputSameDT=on  SaturateOnIntegerOverflow=on  OutDataTypeStr=Inherit: Same as first input
  Reference Length : Gain  Gain=beaver_c  SaturateOnIntegerOverflow=on  OutDataTypeStr=Inherit: Same as input  ParamDataTypeStr=Inherit: Same as input
  Reference Span : Gain  Gain=beaver_b/2  SaturateOnIntegerOverflow=on  OutDataTypeStr=Inherit: Same as input  ParamDataTypeStr=Inherit: Same as input
  "Reference Span " : Gain  Gain=beaver_b/2  SaturateOnIntegerOverflow=on  OutDataTypeStr=Inherit: Same as input  ParamDataTypeStr=Inherit: Same as input
  Sum1 : Sum  Inputs=+++  InputSameDT=on  SaturateOnIntegerOverflow=on  OutDataTypeStr=Inherit: Same as first input
  p : Subsystem
  q : Subsystem
  r : Subsystem
  Coefficients : Outport  VectorParamsAs1DForOutWhenUnconnected=off
  wires:
  p/1(delCoeff) -> Product/1
  q/1(delCoeff) -> Product1/1
  p,q,r/1 -> Demux/1
  Demux/1 -> Product/2  "p"
  Demux/2 -> Product1/2  "q"
  Demux/3 -> Product2/2  "r"
  Sum1/1 -> Display/1, Product3/1
  V/1 -> Product3/2
  Product3/1 -> Coefficients/1
  Product1/1 -> Reference Length/1
  Product2/1 -> "Reference Span "/1
  Product/1 -> Reference Span/1
  r/1(delCoeff) -> Product2/1
  Reference Length/1 -> Sum1/2
  Reference Span/1 -> Display1/1, Sum1/1
  "Reference Span "/1 -> Display2/1, Sum1/3

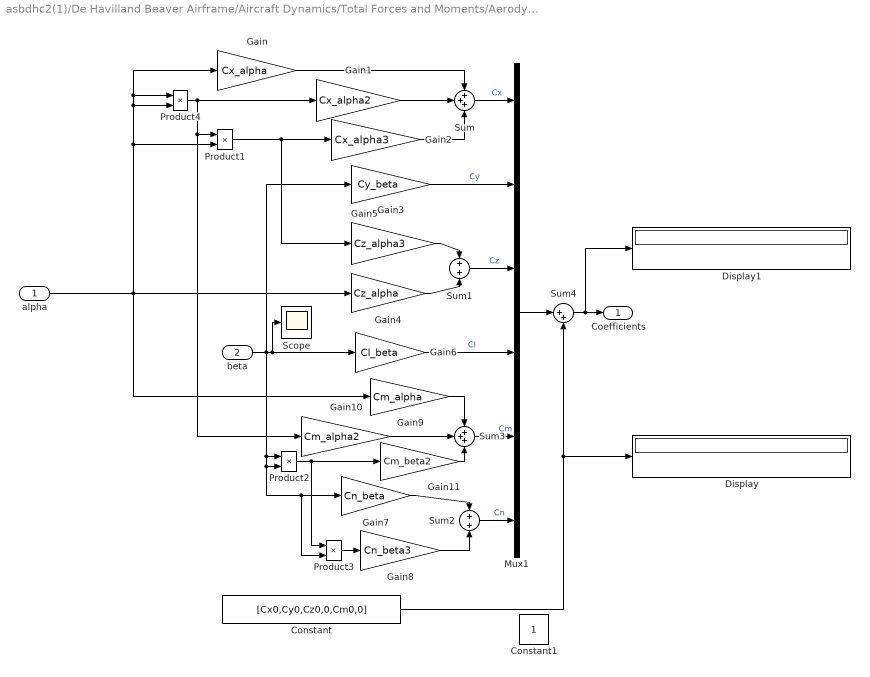
== system asbdhc2(1)/De Havilland Beaver Airframe/Aircraft Dynamics/Total Forces and Moments/Aerodynamics/Datum Coefficients ==
  alpha : Inport  Unit=radian
  beta : Inport  Port=2  Unit=radian
  Constant : Constant  Value=[Cx0,Cy0,Cz0,0,Cm0,0]
  Constant1 : Constant
  Display : Display
  Display1 : Display
  Gain : Gain  Gain=Cx_alpha  SaturateOnIntegerOverflow=on  OutDataTypeStr=Inherit: Same as input  ParamDataTypeStr=Inherit: Same as input
  Gain1 : Gain  Gain=Cx_alpha2  SaturateOnIntegerOverflow=on  OutDataTypeStr=Inherit: Same as input  ParamDataTypeStr=Inherit: Same as input
  Gain10 : Gain  Gain=Cm_alpha2  SaturateOnIntegerOverflow=on  OutDataTypeStr=Inherit: Same as input  ParamDataTypeStr=Inherit: Same as input
  Gain11 : Gain  Gain=Cm_beta2  SaturateOnIntegerOverflow=on  OutDataTypeStr=Inherit: Same as input  ParamDataTypeStr=Inherit: Same as input
  Gain2 : Gain  Gain=Cx_alpha3  SaturateOnIntegerOverflow=on  OutDataTypeStr=Inherit: Same as input  ParamDataTypeStr=Inherit: Same as input
  Gain3 : Gain  Gain=Cy_beta  SaturateOnIntegerOverflow=on  OutDataTypeStr=Inherit: Same as input  ParamDataTypeStr=Inherit: Same as input
  Gain4 : Gain  Gain=Cz_alpha  SaturateOnIntegerOverflow=on  OutDataTypeStr=Inherit: Same as input  ParamDataTypeStr=Inherit: Same as input
  Gain5 : Gain  Gain=Cz_alpha3  SaturateOnIntegerOverflow=on  OutDataTypeStr=Inherit: Same as input  ParamDataTypeStr=Inherit: Same as input
  Gain6 : Gain  Gain=Cl_beta  SaturateOnIntegerOverflow=on  OutDataTypeStr=Inherit: Same as input  ParamDataTypeStr=Inherit: Same as input
  Gain7 : Gain  Gain=Cn_beta  SaturateOnIntegerOverflow=on  OutDataTypeStr=Inherit: Same as input  ParamDataTypeStr=Inherit: Same as input
  Gain8 : Gain  Gain=Cn_beta3  SaturateOnIntegerOverflow=on  OutDataTypeStr=Inherit: Same as input  ParamDataTypeStr=Inherit: Same as input
  Gain9 : Gain  Gain=Cm_alpha  SaturateOnIntegerOverflow=on  OutDataTypeStr=Inherit: Same as input  ParamDataTypeStr=Inherit: Same as input
  Mux1 : Mux  Inputs=6
  Product{1..4} (4 alike) : Product  InputSameDT=on  SaturateOnIntegerOverflow=on  OutDataTypeStr=Inherit: Same as first input
  Scope : Scope
  Sum : Sum  Inputs=+++  SaturateOnIntegerOverflow=on
  Sum1 : Sum  SaturateOnIntegerOverflow=on
  Sum2 : Sum  SaturateOnIntegerOverflow=on
  Sum3 : Sum  Inputs=+++  SaturateOnIntegerOverflow=on
  Sum4 : Sum  Inputs=|++  SaturateOnIntegerOverflow=on
  Coefficients : Outport  VectorParamsAs1DForOutWhenUnconnected=off
  wires:
  Constant/1 -> Sum4/2, Display/1
  Sum4/1 -> Display1/1, Coefficients/1
  Mux1/1 -> Sum4/1
  Gain10/1 -> Sum3/2
  Product2/1 -> Product3/1, Gain11/1
  Gain11/1 -> Sum3/3
  Gain9/1 -> Sum3/1
  Sum3/1 -> Mux1/5  "Cm"
  Product3/1 -> Gain8/1
  Gain8/1 -> Sum2/2
  Gain7/1 -> Sum2/1
  Gain5/1 -> Sum1/1
  Gain4/1 -> Sum1/2
  Product1/1 -> Gain5/1, Gain2/1
  Gain2/1 -> Sum/3
  Product4/1 -> Product1/1, Gain10/1, Gain1/1
  Gain1/1 -> Sum/2
  Gain/1 -> Sum/1
  Sum2/1 -> Mux1/6  "Cn"
  Sum/1 -> Mux1/1  "Cx"
  Sum1/1 -> Mux1/3  "Cz"
  Gain3/1 -> Mux1/2  "Cy"
  Gain6/1 -> Mux1/4  "Cl"
  alpha/1 -> Product1/2, Product4/2, Product4/1, Gain/1, Gain9/1, Gain4/1
  beta/1 -> Scope/1, Gain6/1, Gain3/1, Product3/2, Gain7/1, Product2/2, Product2/1
